simulink model "ForwardKinematic_YuMi"  (R2024a)
(part 17 of 23)

(2579692110316253*sin(q1R))/4503599627370496))/36893488147419103232 + sin(q2R)*((2579692110316253*cos(q1R))/4503599627370496 - (1917820484151683*sin(q1R))/18014398509481984)))/12259964326927110866866776217202473468949912977468817408 + (1764482024691522628700660907665*sin(q3R)*(cos(q2R)*((2579692110316253*cos(q1R))/4503599627370496 - (1917820484151683*sin(q1R))/18014398509481984) - (32968958366167862000829996477285*sin(q2R))/40564819207303340847894502572032 + (7514214926474921*sin(q2R)*((1917820484151683*cos(q1R))/18014398509481984 + (2579692110316253*sin(q1R))/4503599627370496))/36893488147419103232))/42535295865117307932921825928971026432 + (67682029681889335677290557259385*cos(q4R)*(cos(q3R)*(cos(q2R)*((2579692110316253*cos(q1R))/4503599627370496 - (1917820484151683*sin(q1R))/18014398509481984) - (32968958366167862000829996477285*sin(q2R))/40564819207303340847894502572032 + (7514214926474921*sin(q2R)*((1917820484151683*cos(q1R))/18014398509481984 + (2579692110316253*sin(q1R))/4503599627370496))/36893488147419103232) - (9007199067919185*sin(q3R)*((17274190877287359225804725738355*cos(q1R))/162259276829213363391578010288128 + (23235800371559029388956996013805*sin(q1R))/40564819207303340847894502572032 + 27504203825998033884751021716381/166153499473114484112975882535043072))/9007199254740992 + (7514214926474921*sin(q3R)*((32968958366167862000829996477285*cos(q2R))/40564819207303340847894502572032 - (7514214926474921*cos(q2R)*((1917820484151683*cos(q1R))/18014398509481984 + (2579692110316253*sin(q1R))/4503599627370496))/36893488147419103232 + sin(q2R)*((2579692110316253*cos(q1R))/4503599627370496 - (1917820484151683*sin(q1R))/18014398509481984)))/36893488147419103232))/332306998946228968225951765070086144))/16225927682921336339157801028812800 - (2436553109258773196144549622003023*cos(q6R)*(sin(q5R)*(((7514214926474921*cos(q4R))/36893488147419103232 + (4503599440548691*sin(q4R))/4503599627370496)*((9007199067919185*cos(q3R)*((17274190877287359225804725738355*cos(q1R))/162259276829213363391578010288128 + (23235800371559029388956996013805*sin(q1R))/40564819207303340847894502572032 + 27504203825998033884751021716381/166153499473114484112975882535043072))/9007199254740992 - (7514214926474921*cos(q3R)*((32968958366167862000829996477285*cos(q2R))/40564819207303340847894502572032 - (7514214926474921*cos(q2R)*((1917820484151683*cos(q1R))/18014398509481984 + (2579692110316253*sin(q1R))/4503599627370496))/36893488147419103232 + sin(q2R)*((2579692110316253*cos(q1R))/4503599627370496 - (1917820484151683*sin(q1R))/18014398509481984)))/36893488147419103232 + sin(q3R)*(cos(q2R)*((2579692110316253*cos(q1R))/4503599627370496 - (1917820484151683*sin(q1R))/18014398509481984) - (32968958366167862000829996477285*sin(q2R))/40564819207303340847894502572032 + (7514214926474921*sin(q2R)*((1917820484151683*cos(q1R))/18014398509481984 + (2579692110316253*sin(q1R))/4503599627370496))/36893488147419103232)) + (7514214926474921*sin(q4R)*(cos(q3R)*(cos(q2R)*((2579692110316253*cos(q1R))/4503599627370496 - (1917820484151683*sin(q1R))/18014398509481984) - (32968958366167862000829996477285*sin(q2R))/40564819207303340847894502572032 + (7514214926474921*sin(q2R)*((1917820484151683*cos(q1R))/18014398509481984 + (2579692110316253*sin(q1R))/4503599627370496))/36893488147419103232) - (9007199067919185*sin(q3R)*((17274190877287359225804725738355*cos(q1R))/162259276829213363391578010288128 + (23235800371559029388956996013805*sin(q1R))/40564819207303340847894502572032 + 27504203825998033884751021716381/166153499473114484112975882535043072))/9007199254740992 + (7514214926474921*sin(q3R)*((32968958366167862000829996477285*cos(q2R))/40564819207303340847894502572032 - (7514214926474921*cos(q2R)*((1917820484151683*cos(q1R))/18014398509481984 + (2579692110316253*sin(q1R))/4503599627370496))/36893488147419103232 + sin(q2R)*((2579692110316253*cos(q1R))/4503599627370496 - (1917820484151683*sin(q1R))/18014398509481984)))/36893488147419103232))/36893488147419103232) - (9007199067919185*cos(q5R)*((2115063383689692319117831580025*cos(q3R)*((17274190877287359225804725738355*cos(q1R))/162259276829213363391578010288128 + (23235800371559029388956996013805*sin(q1R))/40564819207303340847894502572032 + 27504203825998033884751021716381/166153499473114484112975882535043072))/10384593717069655257060992658440192 + (81129635049124235038645691064225*sin(q3R)*((17274190877287359225804725738355*cos(q1R))/162259276829213363391578010288128 + (23235800371559029388956996013805*sin(q1R))/40564819207303340847894502572032 + 27504203825998033884751021716381/166153499473114484112975882535043072))/81129638414606681695789005144064 - (1764482024691522628700660907665*cos(q3R)*((32968958366167862000829996477285*cos(q2R))/40564819207303340847894502572032 - (7514214926474921*cos(q2R)*((1917820484151683*cos(q1R))/18014398509481984 + (2579692110316253*sin(q1R))/4503599627370496))/36893488147419103232 + sin(q2R)*((2579692110316253*cos(q1R))/4503599627370496 - (1917820484151683*sin(q1R))/18014398509481984)))/42535295865117307932921825928971026432 - (9007199067919185*cos(q3R)*(cos(q2R)*((2579692110316253*cos(q1R))/4503599627370496 - (1917820484151683*sin(q1R))/18014398509481984) - (32968958366167862000829996477285*sin(q2R))/40564819207303340847894502572032 + (7514214926474921*sin(q2R)*((1917820484151683*cos(q1R))/18014398509481984 + (2579692110316253*sin(q1R))/4503599627370496))/36893488147419103232))/9007199254740992 - (67682029681889335677290557259385*sin(q3R)*((32968958366167862000829996477285*cos(q2R))/40564819207303340847894502572032 - (7514214926474921*cos(q2R)*((1917820484151683*cos(q1R))/18014398509481984 + (2579692110316253*sin(q1R))/4503599627370496))/36893488147419103232 + sin(q2R)*((2579692110316253*cos(q1R))/4503599627370496 - (1917820484151683*sin(q1R))/18014398509481984)))/332306998946228968225951765070086144 + (234819211581865*sin(q3R)*(cos(q2R)*((2579692110316253*cos(q1R))/4503599627370496 - (1917820484151683*sin(q1R))/18014398509481984) - (32968958366167862000829996477285*sin(q2R))/40564819207303340847894502572032 + (7514214926474921*sin(q2R)*((1917820484151683*cos(q1R))/18014398509481984 + (2579692110316253*sin(q1R))/4503599627370496))/36893488147419103232))/1152921504606846976))/9007199254740992 + (7514214926474921*cos(q5R)*(((4503599440548691*cos(q4R))/4503599627370496 - (7514214926474921*sin(q4R))/36893488147419103232)*((9007199067919185*cos(q3R)*((17274190877287359225804725738355*cos(q1R))/162259276829213363391578010288128 + (23235800371559029388956996013805*sin(q1R))/40564819207303340847894502572032 + 27504203825998033884751021716381/166153499473114484112975882535043072))/9007199254740992 - (7514214926474921*cos(q3R)*((32968958366167862000829996477285*cos(q2R))/40564819207303340847894502572032 - (7514214926474921*cos(q2R)*((1917820484151683*cos(q1R))/18014398509481984 + (2579692110316253*sin(q1R))/4503599627370496))/36893488147419103232 + sin(q2R)*((2579692110316253*cos(q1R))/4503599627370496 - (1917820484151683*sin(q1R))/18014398509481984)))/36893488147419103232 + sin(q3R)*(cos(q2R)*((2579692110316253*cos(q1R))/4503599627370496 - (1917820484151683*sin(q1R))/18014398509481984) - (32968958366167862000829996477285*sin(q2R))/40564819207303340847894502572032 + (7514214926474921*sin(q2R)*((1917820484151683*cos(q1R))/18014398509481984 + (2579692110316253*sin(q1R))/4503599627370496))/36893488147419103232)) + (7514214926474921*cos(q4R)*(cos(q3R)*(cos(q2R)*((2579692110316253*cos(q1R))/4503599627370496 - (1917820484151683*sin(q1R))/18014398509481984) - (32968958366167862000829996477285*sin(q2R))/40564819207303340847894502572032 + (7514214926474921*sin(q2R)*((1917820484151683*cos(q1R))/18014398509481984 + (2579692110316253*sin(q1R))/4503599627370496))/36893488147419103232) - (9007199067919185*sin(q3R)*((17274190877287359225804725738355*cos(q1R))/162259276829213363391578010288128 + (23235800371559029388956996013805*sin(q1R))/40564819207303340847894502572032 + 27504203825998033884751021716381/166153499473114484112975882535043072))/9007199254740992 + (7514214926474921*sin(q3R)*((32968958366167862000829996477285*cos(q2R))/40564819207303340847894502572032 - (7514214926474921*cos(q2R)*((1917820484151683*cos(q1R))/18014398509481984 + (2579692110316253*sin(q1R))/4503599627370496))/36893488147419103232 + sin(q2R)*((2579692110316253*cos(q1R))/4503599627370496 - (1917820484151683*sin(q1R))/18014398509481984)))/36893488147419103232))/36893488147419103232))/36893488147419103232))/332306998946228968225951765070086144000 - (48638874966763599*sin(q6R)*((15893040848161638993908057577265778144967053025*cos(q3R)*((17274190877287359225804725738355*cos(q1R))/162259276829213363391578010288128 + (23235800371559029388956996013805*sin(q1R))/40564819207303340847894502572032 + 27504203825998033884751021716381/166153499473114484112975882535043072))/383123885216472214589586756787577295904684780545900544 + (609625514665592237562888769449172969868262801225*sin(q3R)*((17274190877287359225804725738355*cos(q1R))/162259276829213363391578010288128 + (23235800371559029388956996013805*sin(q1R))/40564819207303340847894502572032 + 27504203825998033884751021716381/166153499473114484112975882535043072))/2993155353253689176481146537402947624255349848014848 + (9007199067919185*((4503599440548691*cos(q4R))/4503599627370496 - (7514214926474921*sin(q4R))/36893488147419103232)*((9007199067919185*cos(q3R)*((17274190877287359225804725738355*cos(q1R))/162259276829213363391578010288128 + (23235800371559029388956996013805*sin(q1R))/40564819207303340847894502572032 + 27504203825998033884751021716381/166153499473114484112975882535043072))/9007199254740992 - (7514214926474921*cos(q3R)*((32968958366167862000829996477285*cos(q2R))/40564819207303340847894502572032 - (7514214926474921*cos(q2R)*((1917820484151683*cos(q1R))/18014398509481984 + (2579692110316253*sin(q1R))/4503599627370496))/36893488147419103232 + sin(q2R)*((2579692110316253*cos(q1R))/4503599627370496 - (1917820484151683*sin(q1R))/18014398509481984)))/36893488147419103232 + sin(q3R)*(cos(q2R)*((2579692110316253*cos(q1R))/4503599627370496 - (1917820484151683*sin(q1R))/18014398509481984) - (32968958366167862000829996477285*sin(q2R))/40564819207303340847894502572032 + (7514214926474921*sin(q2R)*((1917820484151683*cos(q1R))/18014398509481984 + (2579692110316253*sin(q1R))/4503599627370496))/36893488147419103232)))/9007199254740992 - (13258697167433729449897784796786197386719169465*cos(q3R)*((32968958366167862000829996477285*cos(q2R))/40564819207303340847894502572032 - (7514214926474921*cos(q2R)*((1917820484151683*cos(q1R))/18014398509481984 + (2579692110316253*sin(q1R))/4503599627370496))/36893488147419103232 + sin(q2R)*((2579692110316253*cos(q1R))/4503599627370496 - (1917820484151683*sin(q1R))/18014398509481984)))/1569275433846670190958947355801916604025588861116008628224 - (67682029681889335677290557259385*cos(q3R)*(cos(q2R)*((2579692110316253*cos(q1R))/4503599627370496 - (1917820484151683*sin(q1R))/18014398509481984) - (32968958366167862000829996477285*sin(q2R))/40564819207303340847894502572032 + (7514214926474921*sin(q2R)*((1917820484151683*cos(q1R))/18014398509481984 + (2579692110316253*sin(q1R))/4503599627370496))/36893488147419103232))/332306998946228968225951765070086144 - (508577317689771495245073589786522929324694383585*sin(q3R)*((32968958366167862000829996477285*cos(q2R))/40564819207303340847894502572032 - (7514214926474921*cos(q2R)*((1917820484151683*cos(q1R))/18014398509481984 + (2579692110316253*sin(q1R))/4503599627370496))/36893488147419103232 + sin(q2R)*((2579692110316253*cos(q1R))/4503599627370496 - (1917820484151683*sin(q1R))/18014398509481984)))/12259964326927110866866776217202473468949912977468817408 + (1764482024691522628700660907665*sin(q3R)*(cos(q2R)*((2579692110316253*cos(q1R))/4503599627370496 - (1917820484151683*sin(q1R))/18014398509481984) - (32968958366167862000829996477285*sin(q2R))/40564819207303340847894502572032 + (7514214926474921*sin(q2R)*((1917820484151683*cos(q1R))/18014398509481984 + (2579692110316253*sin(q1R))/4503599627370496))/36893488147419103232))/42535295865117307932921825928971026432 + (67682029681889335677290557259385*cos(q4R)*(cos(q3R)*(cos(q2R)*((2579692110316253*cos(q1R))/4503599627370496 - (1917820484151683*sin(q1R))/18014398509481984) - (32968958366167862000829996477285*sin(q2R))/40564819207303340847894502572032 + (7514214926474921*sin(q2R)*((1917820484151683*cos(q1R))/18014398509481984 + (2579692110316253*sin(q1R))/4503599627370496))/36893488147419103232) - (9007199067919185*sin(q3R)*((17274190877287359225804725738355*cos(q1R))/162259276829213363391578010288128 + (23235800371559029388956996013805*sin(q1R))/40564819207303340847894502572032 + 27504203825998033884751021716381/166153499473114484112975882535043072))/9007199254740992 + (7514214926474921*sin(q3R)*((32968958366167862000829996477285*cos(q2R))/40564819207303340847894502572032 - (7514214926474921*cos(q2R)*((1917820484151683*cos(q1R))/18014398509481984 + (2579692110316253*sin(q1R))/4503599627370496))/36893488147419103232 + sin(q2R)*((2579692110316253*cos(q1R))/4503599627370496 - (1917820484151683*sin(q1R))/18014398509481984)))/36893488147419103232))/332306998946228968225951765070086144))/1801439850948198400 - (27*cos(q6R)*(cos(q5R)*(((7514214926474921*cos(q4R))/36893488147419103232 + (4503599440548691*sin(q4R))/4503599627370496)*((9007199067919185*cos(q3R)*((17274190877287359225804725738355*cos(q1R))/162259276829213363391578010288128 + (23235800371559029388956996013805*sin(q1R))/40564819207303340847894502572032 + 27504203825998033884751021716381/166153499473114484112975882535043072))/9007199254740992 - (7514214926474921*cos(q3R)*((32968958366167862000829996477285*cos(q2R))/40564819207303340847894502572032 - (7514214926474921*cos(q2R)*((1917820484151683*cos(q1R))/18014398509481984 + (2579692110316253*sin(q1R))/4503599627370496))/36893488147419103232 + sin(q2R)*((2579692110316253*cos(q1R))/4503599627370496 - (1917820484151683*sin(q1R))/18014398509481984)))/36893488147419103232 + sin(q3R)*(cos(q2R)*((2579692110316253*cos(q1R))/4503599627370496 - (1917820484151683*sin(q1R))/18014398509481984) - (32968958366167862000829996477285*sin(q2R))/40564819207303340847894502572032 + (7514214926474921*sin(q2R)*((1917820484151683*cos(q1R))/18014398509481984 + (2579692110316253*sin(q1R))/4503599627370496))/36893488147419103232)) + (7514214926474921*sin(q4R)*(cos(q3R)*(cos(q2R)*((2579692110316253*cos(q1R))/4503599627370496 - (1917820484151683*sin(q1R))/18014398509481984) - (32968958366167862000829996477285*sin(q2R))/40564819207303340847894502572032 + (7514214926474921*sin(q2R)*((1917820484151683*cos(q1R))/18014398509481984 + (2579692110316253*sin(q1R))/4503599627370496))/36893488147419103232) - (9007199067919185*sin(q3R)*((17274190877287359225804725738355*cos(q1R))/162259276829213363391578010288128 + (23235800371559029388956996013805*sin(q1R))/40564819207303340847894502572032 + 27504203825998033884751021716381/166153499473114484112975882535043072))/9007199254740992 + (7514214926474921*sin(q3R)*((32968958366167862000829996477285*cos(q2R))/40564819207303340847894502572032 - (7514214926474921*cos(q2R)*((1917820484151683*cos(q1R))/18014398509481984 + (2579692110316253*sin(q1R))/4503599627370496))/36893488147419103232 + sin(q2R)*((2579692110316253*cos(q1R))/4503599627370496 - (1917820484151683*sin(q1R))/18014398509481984)))/36893488147419103232))/36893488147419103232) - (7514214926474921*sin(q5R)*(((4503599440548691*cos(q4R))/4503599627370496 - (7514214926474921*sin(q4R))/36893488147419103232)*((9007199067919185*cos(q3R)*((17274190877287359225804725738355*cos(q1R))/162259276829213363391578010288128 + (23235800371559029388956996013805*sin(q1R))/40564819207303340847894502572032 + 27504203825998033884751021716381/166153499473114484112975882535043072))/9007199254740992 - (7514214926474921*cos(q3R)*((32968958366167862000829996477285*cos(q2R))/40564819207303340847894502572032 - (7514214926474921*cos(q2R)*((1917820484151683*cos(q1R))/18014398509481984 + (2579692110316253*sin(q1R))/4503599627370496))/36893488147419103232 + sin(q2R)*((2579692110316253*cos(q1R))/4503599627370496 - (1917820484151683*sin(q1R))/18014398509481984)))/36893488147419103232 + sin(q3R)*(cos(q2R)*((2579692110316253*cos(q1R))/4503599627370496 - (1917820484151683*sin(q1R))/18014398509481984) - (32968958366167862000829996477285*sin(q2R))/40564819207303340847894502572032 + (7514214926474921*sin(q2R)*((1917820484151683*cos(q1R))/18014398509481984 + (2579692110316253*sin(q1R))/4503599627370496))/36893488147419103232)) + (7514214926474921*cos(q4R)*(cos(q3R)*(cos(q2R)*((2579692110316253*cos(q1R))/4503599627370496 - (1917820484151683*sin(q1R))/18014398509481984) - (32968958366167862000829996477285*sin(q2R))/40564819207303340847894502572032 + (7514214926474921*sin(q2R)*((1917820484151683*cos(q1R))/18014398509481984 + (2579692110316253*sin(q1R))/4503599627370496))/36893488147419103232) - (9007199067919185*sin(q3R)*((17274190877287359225804725738355*cos(q1R))/162259276829213363391578010288128 + (23235800371559029388956996013805*sin(q1R))/40564819207303340847894502572032 + 27504203825998033884751021716381/166153499473114484112975882535043072))/9007199254740992 + (7514214926474921*sin(q3R)*((32968958366167862000829996477285*cos(q2R))/40564819207303340847894502572032 - (7514214926474921*cos(q2R)*((1917820484151683*cos(q1R))/18014398509481984 + (2579692110316253*sin(q1R))/4503599627370496))/36893488147419103232 + sin(q2R)*((2579692110316253*cos(q1R))/4503599627370496 - (1917820484151683*sin(q1R))/18014398509481984)))/36893488147419103232))/36893488147419103232))/36893488147419103232 + (9007199067919185*sin(q5R)*((2115063383689692319117831580025*cos(q3R)*((17274190877287359225804725738355*cos(q1R))/162259276829213363391578010288128 + (23235800371559029388956996013805*sin(q1R))/40564819207303340847894502572032 + 27504203825998033884751021716381/166153499473114484112975882535043072))/10384593717069655257060992658440192 + (81129635049124235038645691064225*sin(q3R)*((17274190877287359225804725738355*cos(q1R))/162259276829213363391578010288128 + (23235800371559029388956996013805*sin(q1R))/40564819207303340847894502572032 + 27504203825998033884751021716381/166153499473114484112975882535043072))/81129638414606681695789005144064 - (1764482024691522628700660907665*cos(q3R)*((32968958366167862000829996477285*cos(q2R))/40564819207303340847894502572032 - (7514214926474921*cos(q2R)*((1917820484151683*cos(q1R))/18014398509481984 + (2579692110316253*sin(q1R))/4503599627370496))/36893488147419103232 + sin(q2R)*((2579692110316253*cos(q1R))/4503599627370496 - (1917820484151683*sin(q1R))/18014398509481984)))/42535295865117307932921825928971026432 - (9007199067919185*cos(q3R)*(cos(q2R)*((2579692110316253*cos(q1R))/4503599627370496 - (1917820484151683*sin(q1R))/18014398509481984) - (32968958366167862000829996477285*sin(q2R))/40564819207303340847894502572032 + (7514214926474921*sin(q2R)*((1917820484151683*cos(q1R))/18014398509481984 + (2579692110316253*sin(q1R))/4503599627370496))/36893488147419103232))/9007199254740992 - (67682029681889335677290557259385*sin(q3R)*((32968958366167862000829996477285*cos(q2R))/40564819207303340847894502572032 - (7514214926474921*cos(q2R)*((1917820484151683*cos(q1R))/18014398509481984 + (2579692110316253*sin(q1R))/4503599627370496))/36893488147419103232 + sin(q2R)*((2579692110316253*cos(q1R))/4503599627370496 - (1917820484151683*sin(q1R))/18014398509481984)))/332306998946228968225951765070086144 + (234819211581865*sin(q3R)*(cos(q2R)*((2579692110316253*cos(q1R))/4503599627370496 - (1917820484151683*sin(q1R))/18014398509481984) - (32968958366167862000829996477285*sin(q2R))/40564819207303340847894502572032 + (7514214926474921*sin(q2R)*((1917820484151683*cos(q1R))/18014398509481984 + (2579692110316253*sin(q1R))/4503599627370496))/36893488147419103232))/1152921504606846976))/9007199254740992))/1000 - (202883803014822867*sin(q6R)*(sin(q5R)*(((7514214926474921*cos(q4R))/36893488147419103232 + (4503599440548691*sin(q4R))/4503599627370496)*((9007199067919185*cos(q3R)*((17274190877287359225804725738355*cos(q1R))/162259276829213363391578010288128 + (23235800371559029388956996013805*sin(q1R))/40564819207303340847894502572032 + 27504203825998033884751021716381/166153499473114484112975882535043072))/9007199254740992 - (7514214926474921*cos(q3R)*((32968958366167862000829996477285*cos(q2R))/40564819207303340847894502572032 - (7514214926474921*cos(q2R)*((1917820484151683*cos(q1R))/18014398509481984 + (2579692110316253*sin(q1R))/4503599627370496))/36893488147419103232 + sin(q2R)*((2579692110316253*cos(q1R))/4503599627370496 - (1917820484151683*sin(q1R))/18014398509481984)))/36893488147419103232 + sin(q3R)*(cos(q2R)*((2579692110316253*cos(q1R))/4503599627370496 - (1917820484151683*sin(q1R))/18014398509481984) - (32968958366167862000829996477285*sin(q2R))/40564819207303340847894502572032 + (7514214926474921*sin(q2R)*((1917820484151683*cos(q1R))/18014398509481984 + (2579692110316253*sin(q1R))/4503599627370496))/36893488147419103232)) + (7514214926474921*sin(q4R)*(cos(q3R)*(cos(q2R)*((2579692110316253*cos(q1R))/4503599627370496 - (1917820484151683*sin(q1R))/18014398509481984) - (32968958366167862000829996477285*sin(q2R))/40564819207303340847894502572032 + (7514214926474921*sin(q2R)*((1917820484151683*cos(q1R))/18014398509481984 + (2579692110316253*sin(q1R))/4503599627370496))/36893488147419103232) - (9007199067919185*sin(q3R)*((17274190877287359225804725738355*cos(q1R))/162259276829213363391578010288128 + (23235800371559029388956996013805*sin(q1R))/40564819207303340847894502572032 + 27504203825998033884751021716381/166153499473114484112975882535043072))/9007199254740992 + (7514214926474921*sin(q3R)*((32968958366167862000829996477285*cos(q2R))/40564819207303340847894502572032 - (7514214926474921*cos(q2R)*((1917820484151683*cos(q1R))/18014398509481984 + (2579692110316253*sin(q1R))/4503599627370496))/36893488147419103232 + sin(q2R)*((2579692110316253*cos(q1R))/4503599627370496 - (1917820484151683*sin(q1R))/18014398509481984)))/36893488147419103232))/36893488147419103232) - (9007199067919185*cos(q5R)*((2115063383689692319117831580025*cos(q3R)*((17274190877287359225804725738355*cos(q1R))/162259276829213363391578010288128 + (23235800371559029388956996013805*sin(q1R))/40564819207303340847894502572032 + 27504203825998033884751021716381/166153499473114484112975882535043072))/10384593717069655257060992658440192 + (81129635049124235038645691064225*sin(q3R)*((17274190877287359225804725738355*cos(q1R))/162259276829213363391578010288128 + (23235800371559029388956996013805*sin(q1R))/40564819207303340847894502572032 + 27504203825998033884751021716381/166153499473114484112975882535043072))/81129638414606681695789005144064 - (1764482024691522628700660907665*cos(q3R)*((32968958366167862000829996477285*cos(q2R))/40564819207303340847894502572032 - (7514214926474921*cos(q2R)*((1917820484151683*cos(q1R))/18014398509481984 + (2579692110316253*sin(q1R))/4503599627370496))/36893488147419103232 + sin(q2R)*((2579692110316253*cos(q1R))/4503599627370496 - (1917820484151683*sin(q1R))/18014398509481984)))/42535295865117307932921825928971026432 - (9007199067919185*cos(q3R)*(cos(q2R)*((2579692110316253*cos(q1R))/4503599627370496 - (1917820484151683*sin(q1R))/18014398509481984) - (32968958366167862000829996477285*sin(q2R))/40564819207303340847894502572032 + (7514214926474921*sin(q2R)*((1917820484151683*cos(q1R))/18014398509481984 + (2579692110316253*sin(q1R))/4503599627370496))/36893488147419103232))/9007199254740992 - (67682029681889335677290557259385*sin(q3R)*((32968958366167862000829996477285*cos(q2R))/40564819207303340847894502572032 - (7514214926474921*cos(q2R)*((1917820484151683*cos(q1R))/18014398509481984 + (2579692110316253*sin(q1R))/4503599627370496))/36893488147419103232 + sin(q2R)*((2579692110316253*cos(q1R))/4503599627370496 - (1917820484151683*sin(q1R))/18014398509481984)))/332306998946228968225951765070086144 + (234819211581865*sin(q3R)*(cos(q2R)*((2579692110316253*cos(q1R))/4503599627370496 - (1917820484151683*sin(q1R))/18014398509481984) - (32968958366167862000829996477285*sin(q2R))/40564819207303340847894502572032 + (7514214926474921*sin(q2R)*((1917820484151683*cos(q1R))/18014398509481984 + (2579692110316253*sin(q1R))/4503599627370496))/36893488147419103232))/1152921504606846976))/9007199254740992 + (7514214926474921*cos(q5R)*(((4503599440548691*cos(q4R))/4503599627370496 - (7514214926474921*sin(q4R))/36893488147419103232)*((9007199067919185*cos(q3R)*((17274190877287359225804725738355*cos(q1R))/162259276829213363391578010288128 + (23235800371559029388956996013805*sin(q1R))/40564819207303340847894502572032 + 27504203825998033884751021716381/166153499473114484112975882535043072))/9007199254740992 - (7514214926474921*cos(q3R)*((32968958366167862000829996477285*cos(q2R))/40564819207303340847894502572032 - (7514214926474921*cos(q2R)*((1917820484151683*cos(q1R))/18014398509481984 + (2579692110316253*sin(q1R))/4503599627370496))/36893488147419103232 + sin(q2R)*((2579692110316253*cos(q1R))/4503599627370496 - (1917820484151683*sin(q1R))/18014398509481984)))/36893488147419103232 + sin(q3R)*(cos(q2R)*((2579692110316253*cos(q1R))/4503599627370496 - (1917820484151683*sin(q1R))/18014398509481984) - (32968958366167862000829996477285*sin(q2R))/40564819207303340847894502572032 + (7514214926474921*sin(q2R)*((1917820484151683*cos(q1R))/18014398509481984 + (2579692110316253*sin(q1R))/4503599627370496))/36893488147419103232)) + (7514214926474921*cos(q4R)*(cos(q3R)*(cos(q2R)*((2579692110316253*cos(q1R))/4503599627370496 - (1917820484151683*sin(q1R))/18014398509481984) - (32968958366167862000829996477285*sin(q2R))/40564819207303340847894502572032 + (7514214926474921*sin(q2R)*((1917820484151683*cos(q1R))/18014398509481984 + (2579692110316253*sin(q1R))/4503599627370496))/36893488147419103232) - (9007199067919185*sin(q3R)*((17274190877287359225804725738355*cos(q1R))/162259276829213363391578010288128 + (23235800371559029388956996013805*sin(q1R))/40564819207303340847894502572032 + 27504203825998033884751021716381/166153499473114484112975882535043072))/9007199254740992 + (7514214926474921*sin(q3R)*((32968958366167862000829996477285*cos(q2R))/40564819207303340847894502572032 - (7514214926474921*cos(q2R)*((1917820484151683*cos(q1R))/18014398509481984 + (2579692110316253*sin(q1R))/4503599627370496))/36893488147419103232 + sin(q2R)*((2579692110316253*cos(q1R))/4503599627370496 - (1917820484151683*sin(q1R))/18014398509481984)))/36893488147419103232))/36893488147419103232))/36893488147419103232))/36893488147419103232000 - (610321541873521657855151997354401418608858870661075444886782706002880706727*cos(q4R)*(cos(q3R)*(cos(q2R)*((2579692110316253*cos(q1R))/4503599627370496 - (1917820484151683*sin(q1R))/18014398509481984) - (32968958366167862000829996477285*sin(q2R))/40564819207303340847894502572032 + (7514214926474921*sin(q2R)*((1917820484151683*cos(q1R))/18014398509481984 + (2579692110316253*sin(q1R))/4503599627370496))/36893488147419103232) - (9007199067919185*sin(q3R)*((17274190877287359225804725738355*cos(q1R))/162259276829213363391578010288128 + (23235800371559029388956996013805*sin(q1R))/40564819207303340847894502572032 + 27504203825998033884751021716381/166153499473114484112975882535043072))/9007199254740992 + (7514214926474921*sin(q3R)*((32968958366167862000829996477285*cos(q2R))/40564819207303340847894502572032 - (7514214926474921*cos(q2R)*((1917820484151683*cos(q1R))/18014398509481984 + (2579692110316253*sin(q1R))/4503599627370496))/36893488147419103232 + sin(q2R)*((2579692110316253*cos(q1R))/4503599627370496 - (1917820484151683*sin(q1R))/18014398509481984)))/36893488147419103232))/11307821214581659709333104004754678501295896940003961331978279688272766566400000 + (324259171862923063*sin(q6R)*(cos(q5R)*(((7514214926474921*cos(q4R))/36893488147419103232 + (4503599440548691*sin(q4R))/4503599627370496)*((9007199067919185*cos(q3R)*((17274190877287359225804725738355*cos(q1R))/162259276829213363391578010288128 + (23235800371559029388956996013805*sin(q1R))/40564819207303340847894502572032 + 27504203825998033884751021716381/166153499473114484112975882535043072))/9007199254740992 - (7514214926474921*cos(q3R)*((32968958366167862000829996477285*cos(q2R))/40564819207303340847894502572032 - (7514214926474921*cos(q2R)*((1917820484151683*cos(q1R))/18014398509481984 + (2579692110316253*sin(q1R))/4503599627370496))/36893488147419103232 + sin(q2R)*((2579692110316253*cos(q1R))/4503599627370496 - (1917820484151683*sin(q1R))/18014398509481984)))/36893488147419103232 + sin(q3R)*(cos(q2R)*((2579692110316253*cos(q1R))/4503599627370496 - (1917820484151683*sin(q1R))/18014398509481984) - (32968958366167862000829996477285*sin(q2R))/40564819207303340847894502572032 + (7514214926474921*sin(q2R)*((1917820484151683*cos(q1R))/18014398509481984 + (2579692110316253*sin(q1R))/4503599627370496))/36893488147419103232)) + (7514214926474921*sin(q4R)*(cos(q3R)*(cos(q2R)*((2579692110316253*cos(q1R))/4503599627370496 - (1917820484151683*sin(q1R))/18014398509481984) - (32968958366167862000829996477285*sin(q2R))/40564819207303340847894502572032 + (7514214926474921*sin(q2R)*((1917820484151683*cos(q1R))/18014398509481984 + (2579692110316253*sin(q1R))/4503599627370496))/36893488147419103232) - (9007199067919185*sin(q3R)*((17274190877287359225804725738355*cos(q1R))/162259276829213363391578010288128 + (23235800371559029388956996013805*sin(q1R))/40564819207303340847894502572032 + 27504203825998033884751021716381/166153499473114484112975882535043072))/9007199254740992 + (7514214926474921*sin(q3R)*((32968958366167862000829996477285*cos(q2R))/40564819207303340847894502572032 - (7514214926474921*cos(q2R)*((1917820484151683*cos(q1R))/18014398509481984 + (2579692110316253*sin(q1R))/4503599627370496))/36893488147419103232 + sin(q2R)*((2579692110316253*cos(q1R))/4503599627370496 - (1917820484151683*sin(q1R))/18014398509481984)))/36893488147419103232))/36893488147419103232) - (7514214926474921*sin(q5R)*(((4503599440548691*cos(q4R))/4503599627370496 - (7514214926474921*sin(q4R))/36893488147419103232)*((9007199067919185*cos(q3R)*((17274190877287359225804725738355*cos(q1R))/162259276829213363391578010288128 + (23235800371559029388956996013805*sin(q1R))/40564819207303340847894502572032 + 27504203825998033884751021716381/166153499473114484112975882535043072))/9007199254740992 - (7514214926474921*cos(q3R)*((32968958366167862000829996477285*cos(q2R))/40564819207303340847894502572032 - (7514214926474921*cos(q2R)*((1917820484151683*cos(q1R))/18014398509481984 + (2579692110316253*sin(q1R))/4503599627370496))/36893488147419103232 + sin(q2R)*((2579692110316253*cos(q1R))/4503599627370496 - (1917820484151683*sin(q1R))/18014398509481984)))/36893488147419103232 + sin(q3R)*(cos(q2R)*((2579692110316253*cos(q1R))/4503599627370496 - (1917820484151683*sin(q1R))/18014398509481984) - (32968958366167862000829996477285*sin(q2R))/40564819207303340847894502572032 + (7514214926474921*sin(q2R)*((1917820484151683*cos(q1R))/18014398509481984 + (2579692110316253*sin(q1R))/4503599627370496))/36893488147419103232)) + (7514214926474921*cos(q4R)*(cos(q3R)*(cos(q2R)*((2579692110316253*cos(q1R))/4503599627370496 - (1917820484151683*sin(q1R))/18014398509481984) - (32968958366167862000829996477285*sin(q2R))/40564819207303340847894502572032 + (7514214926474921*sin(q2R)*((1917820484151683*cos(q1R))/18014398509481984 + (2579692110316253*sin(q1R))/4503599627370496))/36893488147419103232) - (9007199067919185*sin(q3R)*((17274190877287359225804725738355*cos(q1R))/162259276829213363391578010288128 + (23235800371559029388956996013805*sin(q1R))/40564819207303340847894502572032 + 27504203825998033884751021716381/166153499473114484112975882535043072))/9007199254740992 + (7514214926474921*sin(q3R)*((32968958366167862000829996477285*cos(q2R))/40564819207303340847894502572032 - (7514214926474921*cos(q2R)*((1917820484151683*cos(q1R))/18014398509481984 + (2579692110316253*sin(q1R))/4503599627370496))/36893488147419103232 + sin(q2R)*((2579692110316253*cos(q1R))/4503599627370496 - (1917820484151683*sin(q1R))/18014398509481984)))/36893488147419103232))/36893488147419103232))/36893488147419103232 + (9007199067919185*sin(q5R)*((2115063383689692319117831580025*cos(q3R)*((17274190877287359225804725738355*cos(q1R))/162259276829213363391578010288128 + (23235800371559029388956996013805*sin(q1R))/40564819207303340847894502572032 + 27504203825998033884751021716381/166153499473114484112975882535043072))/10384593717069655257060992658440192 + (81129635049124235038645691064225*sin(q3R)*((17274190877287359225804725738355*cos(q1R))/162259276829213363391578010288128 + (23235800371559029388956996013805*sin(q1R))/40564819207303340847894502572032 + 27504203825998033884751021716381/166153499473114484112975882535043072))/81129638414606681695789005144064 - (1764482024691522628700660907665*cos(q3R)*((32968958366167862000829996477285*cos(q2R))/40564819207303340847894502572032 - (7514214926474921*cos(q2R)*((1917820484151683*cos(q1R))/18014398509481984 + (2579692110316253*sin(q1R))/4503599627370496))/36893488147419103232 + sin(q2R)*((2579692110316253*cos(q1R))/4503599627370496 - (1917820484151683*sin(q1R))/18014398509481984)))/42535295865117307932921825928971026432 - (9007199067919185*cos(q3R)*(cos(q2R)*((2579692110316253*cos(q1R))/4503599627370496 - (1917820484151683*sin(q1R))/18014398509481984) - (32968958366167862000829996477285*sin(q2R))/40564819207303340847894502572032 + (7514214926474921*sin(q2R)*((1917820484151683*cos(q1R))/18014398509481984 + (2579692110316253*sin(q1R))/4503599627370496))/36893488147419103232))/9007199254740992 - (67682029681889335677290557259385*sin(q3R)*((32968958366167862000829996477285*cos(q2R))/40564819207303340847894502572032 - (7514214926474921*cos(q2R)*((1917820484151683*cos(q1R))/18014398509481984 + (2579692110316253*sin(q1R))/4503599627370496))/36893488147419103232 + sin(q2R)*((2579692110316253*cos(q1R))/4503599627370496 - (1917820484151683*sin(q1R))/18014398509481984)))/332306998946228968225951765070086144 + (234819211581865*sin(q3R)*(cos(q2R)*((2579692110316253*cos(q1R))/4503599627370496 - (1917820484151683*sin(q1R))/18014398509481984) - (32968958366167862000829996477285*sin(q2R))/40564819207303340847894502572032 + (7514214926474921*sin(q2R)*((1917820484151683*cos(q1R))/18014398509481984 + (2579692110316253*sin(q1R))/4503599627370496))/36893488147419103232))/1152921504606846976))/9007199254740992))/9007199254740992000 - (608651409044468601*sin(q4R)*(cos(q3R)*(cos(q2R)*((2579692110316253*cos(q1R))/4503599627370496 - (1917820484151683*sin(q1R))/18014398509481984) - (32968958366167862000829996477285*sin(q2R))/40564819207303340847894502572032 + (7514214926474921*sin(q2R)*((1917820484151683*cos(q1R))/18014398509481984 + (2579692110316253*sin(q1R))/4503599627370496))/36893488147419103232) - (9007199067919185*sin(q3R)*((17274190877287359225804725738355*cos(q1R))/162259276829213363391578010288128 + (23235800371559029388956996013805*sin(q1R))/40564819207303340847894502572032 + 27504203825998033884751021716381/166153499473114484112975882535043072))/9007199254740992 + (7514214926474921*sin(q3R)*((32968958366167862000829996477285*cos(q2R))/40564819207303340847894502572032 - (7514214926474921*cos(q2R)*((1917820484151683*cos(q1R))/18014398509481984 + (2579692110316253*sin(q1R))/4503599627370496))/36893488147419103232 + sin(q2R)*((2579692110316253*cos(q1R))/4503599627370496 - (1917820484151683*sin(q1R))/18014398509481984)))/36893488147419103232))/73786976294838206464000 + (712008244765680093343103025701132101054572137019*cos(q5R)*(((4503599440548691*cos(q4R))/4503599627370496 - (7514214926474921*sin(q4R))/36893488147419103232)*((9007199067919185*cos(q3R)*((17274190877287359225804725738355*cos(q1R))/162259276829213363391578010288128 + (23235800371559029388956996013805*sin(q1R))/40564819207303340847894502572032 + 27504203825998033884751021716381/166153499473114484112975882535043072))/9007199254740992 - (7514214926474921*cos(q3R)*((32968958366167862000829996477285*cos(q2R))/40564819207303340847894502572032 - (7514214926474921*cos(q2R)*((1917820484151683*cos(q1R))/18014398509481984 + (2579692110316253*sin(q1R))/4503599627370496))/36893488147419103232 + sin(q2R)*((2579692110316253*cos(q1R))/4503599627370496 - (1917820484151683*sin(q1R))/18014398509481984)))/36893488147419103232 + sin(q3R)*(cos(q2R)*((2579692110316253*cos(q1R))/4503599627370496 - (1917820484151683*sin(q1R))/18014398509481984) - (32968958366167862000829996477285*sin(q2R))/40564819207303340847894502572032 + (7514214926474921*sin(q2R)*((1917820484151683*cos(q1R))/18014398509481984 + (2579692110316253*sin(q1R))/4503599627370496))/36893488147419103232)) + (7514214926474921*cos(q4R)*(cos(q3R)*(cos(q2R)*((2579692110316253*cos(q1R))/4503599627370496 - (1917820484151683*sin(q1R))/18014398509481984) - (32968958366167862000829996477285*sin(q2R))/40564819207303340847894502572032 + (7514214926474921*sin(q2R)*((1917820484151683*cos(q1R))/18014398509481984 + (2579692110316253*sin(q1R))/4503599627370496))/36893488147419103232) - (9007199067919185*sin(q3R)*((17274190877287359225804725738355*cos(q1R))/162259276829213363391578010288128 + (23235800371559029388956996013805*sin(q1R))/40564819207303340847894502572032 + 27504203825998033884751021716381/166153499473114484112975882535043072))/9007199254740992 + (7514214926474921*sin(q3R)*((32968958366167862000829996477285*cos(q2R))/40564819207303340847894502572032 - (7514214926474921*cos(q2R)*((1917820484151683*cos(q1R))/18014398509481984 + (2579692110316253*sin(q1R))/4503599627370496))/36893488147419103232 + sin(q2R)*((2579692110316253*cos(q1R))/4503599627370496 - (1917820484151683*sin(q1R))/18014398509481984)))/36893488147419103232))/36893488147419103232))/2451992865385422173373355243440494693789982595493763481600, (81*((4503599440548691*cos(q4R))/4503599627370496 - (7514214926474921*sin(q4R))/36893488147419103232)*(cos(q3R)*(cos(q2R)*((2579692110316253*cos(q1R))/4503599627370496 - (1917820484151683*sin(q1R))/18014398509481984) - (32968958366167862000829996477285*sin(q2R))/40564819207303340847894502572032 + (7514214926474921*sin(q2R)*((1917820484151683*cos(q1R))/18014398509481984 + (2579692110316253*sin(q1R))/4503599627370496))/36893488147419103232) - (9007199067919185*sin(q3R)*((17274190877287359225804725738355*cos(q1R))/162259276829213363391578010288128 + (23235800371559029388956996013805*sin(q1R))/40564819207303340847894502572032 + 27504203825998033884751021716381/166153499473114484112975882535043072))/9007199254740992 + (7514214926474921*sin(q3R)*((32968958366167862000829996477285*cos(q2R))/40564819207303340847894502572032 - (7514214926474921*cos(q2R)*((1917820484151683*cos(q1R))/18014398509481984 + (2579692110316253*sin(q1R))/4503599627370496))/36893488147419103232 + sin(q2R)*((2579692110316253*cos(q1R))/4503599627370496 - (1917820484151683*sin(q1R))/18014398509481984)))/36893488147419103232))/2000 - (81222263116692158804177042061221826384594597321566869716687*((7514214926474921*cos(q4R))/36893488147419103232 + (4503599440548691*sin(q4R))/4503599627370496)*(cos(q3R)*(cos(q2R)*((2579692110316253*cos(q1R))/4503599627370496 - (1917820484151683*sin(q1R))/18014398509481984) - (32968958366167862000829996477285*sin(q2R))/40564819207303340847894502572032 + (7514214926474921*sin(q2R)*((1917820484151683*cos(q1R))/18014398509481984 + (2579692110316253*sin(q1R))/4503599627370496))/36893488147419103232) - (9007199067919185*sin(q3R)*((17274190877287359225804725738355*cos(q1R))/162259276829213363391578010288128 + (23235800371559029388956996013805*sin(q1R))/40564819207303340847894502572032 + 27504203825998033884751021716381/166153499473114484112975882535043072))/9007199254740992 + (7514214926474921*sin(q3R)*((32968958366167862000829996477285*cos(q2R))/40564819207303340847894502572032 - (7514214926474921*cos(q2R)*((1917820484151683*cos(q1R))/18014398509481984 + (2579692110316253*sin(q1R))/4503599627370496))/36893488147419103232 + sin(q2R)*((2579692110316253*cos(q1R))/4503599627370496 - (1917820484151683*sin(q1R))/18014398509481984)))/36893488147419103232))/306499108173177771671669405430061836723747824436720435200000 - (584133382113593486367040631332731*cos(q6R)*((9007199067919185*((7514214926474921*cos(q4R))/36893488147419103232 + (4503599440548691*sin(q4R))/4503599627370496)*(cos(q3R)*(cos(q2R)*((2579692110316253*cos(q1R))/4503599627370496 - (1917820484151683*sin(q1R))/18014398509481984) - (32968958366167862000829996477285*sin(q2R))/40564819207303340847894502572032 + (7514214926474921*sin(q2R)*((1917820484151683*cos(q1R))/18014398509481984 + (2579692110316253*sin(q1R))/4503599627370496))/36893488147419103232) - (9007199067919185*sin(q3R)*((17274190877287359225804725738355*cos(q1R))/162259276829213363391578010288128 + (23235800371559029388956996013805*sin(q1R))/40564819207303340847894502572032 + 27504203825998033884751021716381/166153499473114484112975882535043072))/9007199254740992 + (7514214926474921*sin(q3R)*((32968958366167862000829996477285*cos(q2R))/40564819207303340847894502572032 - (7514214926474921*cos(q2R)*((1917820484151683*cos(q1R))/18014398509481984 + (2579692110316253*sin(q1R))/4503599627370496))/36893488147419103232 + sin(q2R)*((2579692110316253*cos(q1R))/4503599627370496 - (1917820484151683*sin(q1R))/18014398509481984)))/36893488147419103232))/9007199254740992 - (67682029681889335677290557259385*sin(q4R)*((9007199067919185*cos(q3R)*((17274190877287359225804725738355*cos(q1R))/162259276829213363391578010288128 + (23235800371559029388956996013805*sin(q1R))/40564819207303340847894502572032 + 27504203825998033884751021716381/166153499473114484112975882535043072))/9007199254740992 - (7514214926474921*cos(q3R)*((32968958366167862000829996477285*cos(q2R))/40564819207303340847894502572032 - (7514214926474921*cos(q2R)*((1917820484151683*cos(q1R))/18014398509481984 + (2579692110316253*sin(q1R))/4503599627370496))/36893488147419103232 + sin(q2R)*((2579692110316253*cos(q1R))/4503599627370496 - (1917820484151683*sin(q1R))/18014398509481984)))/36893488147419103232 + sin(q3R)*(cos(q2R)*((2579692110316253*cos(q1R))/4503599627370496 - (1917820484151683*sin(q1R))/18014398509481984) - (32968958366167862000829996477285*sin(q2R))/40564819207303340847894502572032 + (7514214926474921*sin(q2R)*((1917820484151683*cos(q1R))/18014398509481984 + (2579692110316253*sin(q1R))/4503599627370496))/36893488147419103232)))/332306998946228968225951765070086144 + (9007199067919185*((9007199067919185*cos(q4R))/9007199254740992 - (234819211581865*sin(q4R))/1152921504606846976)*((129801982932889585091297864435361917839115294955*cos(q1R))/5986310706507378352962293074805895248510699696029696 + (296957971066013582975066703729047659005068212725*cos(q2R))/365375409332725729550921208179070754913983135744 + (174598797980560374072834504815488878557302284405*sin(q1R))/1496577676626844588240573268701473812127674924007424 - (67682029681889335677290557259385*cos(q2R)*((1917820484151683*cos(q1R))/18014398509481984 + (2579692110316253*sin(q1R))/4503599627370496))/332306998946228968225951765070086144 + (9007199067919185*sin(q2R)*((2579692110316253*cos(q1R))/4503599627370496 - (1917820484151683*sin(q1R))/18014398509481984))/9007199254740992 + 206672498930123057048696703425560088887371380901/6129982163463555433433388108601236734474956488734408704))/9007199254740992))/16225927682921336339157801028812800 - (48638874966763599*sin(q6R)*((9007199067919185*((7514214926474921*cos(q4R))/36893488147419103232 + (4503599440548691*sin(q4R))/4503599627370496)*(cos(q3R)*(cos(q2R)*((2579692110316253*cos(q1R))/4503599627370496 - (1917820484151683*sin(q1R))/18014398509481984) - (32968958366167862000829996477285*sin(q2R))/40564819207303340847894502572032 + (7514214926474921*sin(q2R)*((1917820484151683*cos(q1R))/18014398509481984 + (2579692110316253*sin(q1R))/4503599627370496))/36893488147419103232) - (9007199067919185*sin(q3R)*((17274190877287359225804725738355*cos(q1R))/162259276829213363391578010288128 + (23235800371559029388956996013805*sin(q1R))/40564819207303340847894502572032 + 27504203825998033884751021716381/166153499473114484112975882535043072))/9007199254740992 + (7514214926474921*sin(q3R)*((32968958366167862000829996477285*cos(q2R))/40564819207303340847894502572032 - (7514214926474921*cos(q2R)*((1917820484151683*cos(q1R))/18014398509481984 + (2579692110316253*sin(q1R))/4503599627370496))/36893488147419103232 + sin(q2R)*((2579692110316253*cos(q1R))/4503599627370496 - (1917820484151683*sin(q1R))/18014398509481984)))/36893488147419103232))/9007199254740992 - (67682029681889335677290557259385*sin(q4R)*((9007199067919185*cos(q3R)*((17274190877287359225804725738355*cos(q1R))/162259276829213363391578010288128 + (23235800371559029388956996013805*sin(q1R))/40564819207303340847894502572032 + 27504203825998033884751021716381/166153499473114484112975882535043072))/9007199254740992 - (7514214926474921*cos(q3R)*((32968958366167862000829996477285*cos(q2R))/40564819207303340847894502572032 - (7514214926474921*cos(q2R)*((1917820484151683*cos(q1R))/18014398509481984 + (2579692110316253*sin(q1R))/4503599627370496))/36893488147419103232 + sin(q2R)*((2579692110316253*cos(q1R))/4503599627370496 - (1917820484151683*sin(q1R))/18014398509481984)))/36893488147419103232 + sin(q3R)*(cos(q2R)*((2579692110316253*cos(q1R))/4503599627370496 - (1917820484151683*sin(q1R))/18014398509481984) - (32968958366167862000829996477285*sin(q2R))/40564819207303340847894502572032 + (7514214926474921*sin(q2R)*((1917820484151683*cos(q1R))/18014398509481984 + (2579692110316253*sin(q1R))/4503599627370496))/36893488147419103232)))/332306998946228968225951765070086144 + (9007199067919185*((9007199067919185*cos(q4R))/9007199254740992 - (234819211581865*sin(q4R))/1152921504606846976)*((129801982932889585091297864435361917839115294955*cos(q1R))/5986310706507378352962293074805895248510699696029696 + (296957971066013582975066703729047659005068212725*cos(q2R))/365375409332725729550921208179070754913983135744 + (174598797980560374072834504815488878557302284405*sin(q1R))/1496577676626844588240573268701473812127674924007424 - (67682029681889335677290557259385*cos(q2R)*((1917820484151683*cos(q1R))/18014398509481984 + (2579692110316253*sin(q1R))/4503599627370496))/332306998946228968225951765070086144 + (9007199067919185*sin(q2R)*((2579692110316253*cos(q1R))/4503599627370496 - (1917820484151683*sin(q1R))/18014398509481984))/9007199254740992 + 206672498930123057048696703425560088887371380901/6129982163463555433433388108601236734474956488734408704))/9007199254740992))/1801439850948198400 - (608651409044468601*cos(q4R)*((9007199067919185*cos(q3R)*((17274190877287359225804725738355*cos(q1R))/162259276829213363391578010288128 + (23235800371559029388956996013805*sin(q1R))/40564819207303340847894502572032 + 27504203825998033884751021716381/166153499473114484112975882535043072))/9007199254740992 - (7514214926474921*cos(q3R)*((32968958366167862000829996477285*cos(q2R))/40564819207303340847894502572032 - (7514214926474921*cos(q2R)*((1917820484151683*cos(q1R))/18014398509481984 + (2579692110316253*sin(q1R))/4503599627370496))/36893488147419103232 + sin(q2R)*((2579692110316253*cos(q1R))/4503599627370496 - (1917820484151683*sin(q1R))/18014398509481984)))/36893488147419103232 + sin(q3R)*(cos(q2R)*((2579692110316253*cos(q1R))/4503599627370496 - (1917820484151683*sin(q1R))/18014398509481984) - (32968958366167862000829996477285*sin(q2R))/40564819207303340847894502572032 + (7514214926474921*sin(q2R)*((1917820484151683*cos(q1R))/18014398509481984 + (2579692110316253*sin(q1R))/4503599627370496))/36893488147419103232)))/73786976294838206464000 - (27*cos(q6R)*(cos(q5R)*((7514214926474921*cos(q4R)*((9007199067919185*cos(q3R)*((17274190877287359225804725738355*cos(q1R))/162259276829213363391578010288128 + (23235800371559029388956996013805*sin(q1R))/40564819207303340847894502572032 + 27504203825998033884751021716381/166153499473114484112975882535043072))/9007199254740992 - (7514214926474921*cos(q3R)*((32968958366167862000829996477285*cos(q2R))/40564819207303340847894502572032 - (7514214926474921*cos(q2R)*((1917820484151683*cos(q1R))/18014398509481984 + (2579692110316253*sin(q1R))/4503599627370496))/36893488147419103232 + sin(q2R)*((2579692110316253*cos(q1R))/4503599627370496 - (1917820484151683*sin(q1R))/18014398509481984)))/36893488147419103232 + sin(q3R)*(cos(q2R)*((2579692110316253*cos(q1R))/4503599627370496 - (1917820484151683*sin(q1R))/18014398509481984) - (32968958366167862000829996477285*sin(q2R))/40564819207303340847894502572032 + (7514214926474921*sin(q2R)*((1917820484151683*cos(q1R))/18014398509481984 + (2579692110316253*sin(q1R))/4503599627370496))/36893488147419103232)))/36893488147419103232 - ((4503599440548691*cos(q4R))/4503599627370496 - (7514214926474921*sin(q4R))/36893488147419103232)*(cos(q3R)*(cos(q2R)*((2579692110316253*cos(q1R))/4503599627370496 - (1917820484151683*sin(q1R))/18014398509481984) - (32968958366167862000829996477285*sin(q2R))/40564819207303340847894502572032 + (7514214926474921*sin(q2R)*((1917820484151683*cos(q1R))/18014398509481984 + (2579692110316253*sin(q1R))/4503599627370496))/36893488147419103232) - (9007199067919185*sin(q3R)*((17274190877287359225804725738355*cos(q1R))/162259276829213363391578010288128 + (23235800371559029388956996013805*sin(q1R))/40564819207303340847894502572032 + 27504203825998033884751021716381/166153499473114484112975882535043072))/9007199254740992 + (7514214926474921*sin(q3R)*((32968958366167862000829996477285*cos(q2R))/40564819207303340847894502572032 - (7514214926474921*cos(q2R)*((1917820484151683*cos(q1R))/18014398509481984 + (2579692110316253*sin(q1R))/4503599627370496))/36893488147419103232 + sin(q2R)*((2579692110316253*cos(q1R))/4503599627370496 - (1917820484151683*sin(q1R))/18014398509481984)))/36893488147419103232) + ((234819211581865*cos(q4R))/1152921504606846976 + (9007199067919185*sin(q4R))/9007199254740992)*((129801982932889585091297864435361917839115294955*cos(q1R))/5986310706507378352962293074805895248510699696029696 + (296957971066013582975066703729047659005068212725*cos(q2R))/365375409332725729550921208179070754913983135744 + (174598797980560374072834504815488878557302284405*sin(q1R))/1496577676626844588240573268701473812127674924007424 - (67682029681889335677290557259385*cos(q2R)*((1917820484151683*cos(q1R))/18014398509481984 + (2579692110316253*sin(q1R))/4503599627370496))/332306998946228968225951765070086144 + (9007199067919185*sin(q2R)*((2579692110316253*cos(q1R))/4503599627370496 - (1917820484151683*sin(q1R))/18014398509481984))/9007199254740992 + 206672498930123057048696703425560088887371380901/6129982163463555433433388108601236734474956488734408704)) - (7514214926474921*sin(q5R)*(((7514214926474921*cos(q4R))/36893488147419103232 + (4503599440548691*sin(q4R))/4503599627370496)*(cos(q3R)*(cos(q2R)*((2579692110316253*cos(q1R))/4503599627370496 - (1917820484151683*sin(q1R))/18014398509481984) - (32968958366167862000829996477285*sin(q2R))/40564819207303340847894502572032 + (7514214926474921*sin(q2R)*((1917820484151683*cos(q1R))/18014398509481984 + (2579692110316253*sin(q1R))/4503599627370496))/36893488147419103232) - (9007199067919185*sin(q3R)*((17274190877287359225804725738355*cos(q1R))/162259276829213363391578010288128 + (23235800371559029388956996013805*sin(q1R))/40564819207303340847894502572032 + 27504203825998033884751021716381/166153499473114484112975882535043072))/9007199254740992 + (7514214926474921*sin(q3R)*((32968958366167862000829996477285*cos(q2R))/40564819207303340847894502572032 - (7514214926474921*cos(q2R)*((1917820484151683*cos(q1R))/18014398509481984 + (2579692110316253*sin(q1R))/4503599627370496))/36893488147419103232 + sin(q2R)*((2579692110316253*cos(q1R))/4503599627370496 - (1917820484151683*sin(q1R))/18014398509481984)))/36893488147419103232) - (7514214926474921*sin(q4R)*((9007199067919185*cos(q3R)*((17274190877287359225804725738355*cos(q1R))/162259276829213363391578010288128 + (23235800371559029388956996013805*sin(q1R))/40564819207303340847894502572032 + 27504203825998033884751021716381/166153499473114484112975882535043072))/9007199254740992 - (7514214926474921*cos(q3R)*((32968958366167862000829996477285*cos(q2R))/40564819207303340847894502572032 - (7514214926474921*cos(q2R)*((1917820484151683*cos(q1R))/18014398509481984 + (2579692110316253*sin(q1R))/4503599627370496))/36893488147419103232 + sin(q2R)*((2579692110316253*cos(q1R))/4503599627370496 - (1917820484151683*sin(q1R))/18014398509481984)))/36893488147419103232 + sin(q3R)*(cos(q2R)*((2579692110316253*cos(q1R))/4503599627370496 - (1917820484151683*sin(q1R))/18014398509481984) - (32968958366167862000829996477285*sin(q2R))/40564819207303340847894502572032 + (7514214926474921*sin(q2R)*((1917820484151683*cos(q1R))/18014398509481984 + (2579692110316253*sin(q1R))/4503599627370496))/36893488147419103232)))/36893488147419103232 + ((9007199067919185*cos(q4R))/9007199254740992 - (234819211581865*sin(q4R))/1152921504606846976)*((129801982932889585091297864435361917839115294955*cos(q1R))/5986310706507378352962293074805895248510699696029696 + (296957971066013582975066703729047659005068212725*cos(q2R))/365375409332725729550921208179070754913983135744 + (174598797980560374072834504815488878557302284405*sin(q1R))/1496577676626844588240573268701473812127674924007424 - (67682029681889335677290557259385*cos(q2R)*((1917820484151683*cos(q1R))/18014398509481984 + (2579692110316253*sin(q1R))/4503599627370496))/332306998946228968225951765070086144 + (9007199067919185*sin(q2R)*((2579692110316253*cos(q1R))/4503599627370496 - (1917820484151683*sin(q1R))/18014398509481984))/9007199254740992 + 206672498930123057048696703425560088887371380901/6129982163463555433433388108601236734474956488734408704)))/36893488147419103232))/1000 - (2436553109258773196144549622003023*cos(q6R)*((7514214926474921*cos(q5R)*(((7514214926474921*cos(q4R))/36893488147419103232 + (4503599440548691*sin(q4R))/4503599627370496)*(cos(q3R)*(cos(q2R)*((2579692110316253*cos(q1R))/4503599627370496 - (1917820484151683*sin(q1R))/18014398509481984) - (32968958366167862000829996477285*sin(q2R))/40564819207303340847894502572032 + (7514214926474921*sin(q2R)*((1917820484151683*cos(q1R))/18014398509481984 + (2579692110316253*sin(q1R))/4503599627370496))/36893488147419103232) - (9007199067919185*sin(q3R)*((17274190877287359225804725738355*cos(q1R))/162259276829213363391578010288128 + (23235800371559029388956996013805*sin(q1R))/40564819207303340847894502572032 + 27504203825998033884751021716381/166153499473114484112975882535043072))/9007199254740992 + (7514214926474921*sin(q3R)*((32968958366167862000829996477285*cos(q2R))/40564819207303340847894502572032 - (7514214926474921*cos(q2R)*((1917820484151683*cos(q1R))/18014398509481984 + (2579692110316253*sin(q1R))/4503599627370496))/36893488147419103232 + sin(q2R)*((2579692110316253*cos(q1R))/4503599627370496 - (1917820484151683*sin(q1R))/18014398509481984)))/36893488147419103232) - (7514214926474921*sin(q4R)*((9007199067919185*cos(q3R)*((17274190877287359225804725738355*cos(q1R))/162259276829213363391578010288128 + (23235800371559029388956996013805*sin(q1R))/40564819207303340847894502572032 + 27504203825998033884751021716381/166153499473114484112975882535043072))/9007199254740992 - (7514214926474921*cos(q3R)*((32968958366167862000829996477285*cos(q2R))/40564819207303340847894502572032 - (7514214926474921*cos(q2R)*((1917820484151683*cos(q1R))/18014398509481984 + (2579692110316253*sin(q1R))/4503599627370496))/36893488147419103232 + sin(q2R)*((2579692110316253*cos(q1R))/4503599627370496 - (1917820484151683*sin(q1R))/18014398509481984)))/36893488147419103232 + sin(q3R)*(cos(q2R)*((2579692110316253*cos(q1R))/4503599627370496 - (1917820484151683*sin(q1R))/18014398509481984) - (32968958366167862000829996477285*sin(q2R))/40564819207303340847894502572032 + (7514214926474921*sin(q2R)*((1917820484151683*cos(q1R))/18014398509481984 + (2579692110316253*sin(q1R))/4503599627370496))/36893488147419103232)))/36893488147419103232 + ((9007199067919185*cos(q4R))/9007199254740992 - (234819211581865*sin(q4R))/1152921504606846976)*((129801982932889585091297864435361917839115294955*cos(q1R))/5986310706507378352962293074805895248510699696029696 + (296957971066013582975066703729047659005068212725*cos(q2R))/365375409332725729550921208179070754913983135744 + (174598797980560374072834504815488878557302284405*sin(q1R))/1496577676626844588240573268701473812127674924007424 - (67682029681889335677290557259385*cos(q2R)*((1917820484151683*cos(q1R))/18014398509481984 + (2579692110316253*sin(q1R))/4503599627370496))/332306998946228968225951765070086144 + (9007199067919185*sin(q2R)*((2579692110316253*cos(q1R))/4503599627370496 - (1917820484151683*sin(q1R))/18014398509481984))/9007199254740992 + 206672498930123057048696703425560088887371380901/6129982163463555433433388108601236734474956488734408704)))/36893488147419103232 + sin(q5R)*((7514214926474921*cos(q4R)*((9007199067919185*cos(q3R)*((17274190877287359225804725738355*cos(q1R))/162259276829213363391578010288128 + (23235800371559029388956996013805*sin(q1R))/40564819207303340847894502572032 + 27504203825998033884751021716381/166153499473114484112975882535043072))/9007199254740992 - (7514214926474921*cos(q3R)*((32968958366167862000829996477285*cos(q2R))/40564819207303340847894502572032 - (7514214926474921*cos(q2R)*((1917820484151683*cos(q1R))/18014398509481984 + (2579692110316253*sin(q1R))/4503599627370496))/36893488147419103232 + sin(q2R)*((2579692110316253*cos(q1R))/4503599627370496 - (1917820484151683*sin(q1R))/18014398509481984)))/36893488147419103232 + sin(q3R)*(cos(q2R)*((2579692110316253*cos(q1R))/4503599627370496 - (1917820484151683*sin(q1R))/18014398509481984) - (32968958366167862000829996477285*sin(q2R))/40564819207303340847894502572032 + (7514214926474921*sin(q2R)*((1917820484151683*cos(q1R))/18014398509481984 + (2579692110316253*sin(q1R))/4503599627370496))/36893488147419103232)))/36893488147419103232 - ((4503599440548691*cos(q4R))/4503599627370496 - (7514214926474921*sin(q4R))/36893488147419103232)*(cos(q3R)*(cos(q2R)*((2579692110316253*cos(q1R))/4503599627370496 - (1917820484151683*sin(q1R))/18014398509481984) - (32968958366167862000829996477285*sin(q2R))/40564819207303340847894502572032 + (7514214926474921*sin(q2R)*((1917820484151683*cos(q1R))/18014398509481984 + (2579692110316253*sin(q1R))/4503599627370496))/36893488147419103232) - (9007199067919185*sin(q3R)*((17274190877287359225804725738355*cos(q1R))/162259276829213363391578010288128 + (23235800371559029388956996013805*sin(q1R))/40564819207303340847894502572032 + 27504203825998033884751021716381/166153499473114484112975882535043072))/9007199254740992 + (7514214926474921*sin(q3R)*((32968958366167862000829996477285*cos(q2R))/40564819207303340847894502572032 - (7514214926474921*cos(q2R)*((1917820484151683*cos(q1R))/18014398509481984 + (2579692110316253*sin(q1R))/4503599627370496))/36893488147419103232 + sin(q2R)*((2579692110316253*cos(q1R))/4503599627370496 - (1917820484151683*sin(q1R))/18014398509481984)))/36893488147419103232) + ((234819211581865*cos(q4R))/1152921504606846976 + (9007199067919185*sin(q4R))/9007199254740992)*((129801982932889585091297864435361917839115294955*cos(q1R))/5986310706507378352962293074805895248510699696029696 + (296957971066013582975066703729047659005068212725*cos(q2R))/365375409332725729550921208179070754913983135744 + (174598797980560374072834504815488878557302284405*sin(q1R))/1496577676626844588240573268701473812127674924007424 - (67682029681889335677290557259385*cos(q2R)*((1917820484151683*cos(q1R))/18014398509481984 + (2579692110316253*sin(q1R))/4503599627370496))/332306998946228968225951765070086144 + (9007199067919185*sin(q2R)*((2579692110316253*cos(q1R))/4503599627370496 - (1917820484151683*sin(q1R))/18014398509481984))/9007199254740992 + 206672498930123057048696703425560088887371380901/6129982163463555433433388108601236734474956488734408704))))/332306998946228968225951765070086144000 + (27*cos(q5R)*((7514214926474921*cos(q4R)*((9007199067919185*cos(q3R)*((17274190877287359225804725738355*cos(q1R))/162259276829213363391578010288128 + (23235800371559029388956996013805*sin(q1R))/40564819207303340847894502572032 + 27504203825998033884751021716381/166153499473114484112975882535043072))/9007199254740992 - (7514214926474921*cos(q3R)*((32968958366167862000829996477285*cos(q2R))/40564819207303340847894502572032 - (7514214926474921*cos(q2R)*((1917820484151683*cos(q1R))/18014398509481984 + (2579692110316253*sin(q1R))/4503599627370496))/36893488147419103232 + sin(q2R)*((2579692110316253*cos(q1R))/4503599627370496 - (1917820484151683*sin(q1R))/18014398509481984)))/36893488147419103232 + sin(q3R)*(cos(q2R)*((2579692110316253*cos(q1R))/4503599627370496 - (1917820484151683*sin(q1R))/18014398509481984) - (32968958366167862000829996477285*sin(q2R))/40564819207303340847894502572032 + (7514214926474921*sin(q2R)*((1917820484151683*cos(q1R))/18014398509481984 + (2579692110316253*sin(q1R))/4503599627370496))/36893488147419103232)))/36893488147419103232 - ((4503599440548691*cos(q4R))/4503599627370496 - (7514214926474921*sin(q4R))/36893488147419103232)*(cos(q3R)*(cos(q2R)*((2579692110316253*cos(q1R))/4503599627370496 - (1917820484151683*sin(q1R))/18014398509481984) - (32968958366167862000829996477285*sin(q2R))/40564819207303340847894502572032 + (7514214926474921*sin(q2R)*((1917820484151683*cos(q1R))/18014398509481984 + (2579692110316253*sin(q1R))/4503599627370496))/36893488147419103232) - (9007199067919185*sin(q3R)*((17274190877287359225804725738355*cos(q1R))/162259276829213363391578010288128 + (23235800371559029388956996013805*sin(q1R))/40564819207303340847894502572032 + 27504203825998033884751021716381/166153499473114484112975882535043072))/9007199254740992 + (7514214926474921*sin(q3R)*((32968958366167862000829996477285*cos(q2R))/40564819207303340847894502572032 - (7514214926474921*cos(q2R)*((1917820484151683*cos(q1R))/18014398509481984 + (2579692110316253*sin(q1R))/4503599627370496))/36893488147419103232 + sin(q2R)*((2579692110316253*cos(q1R))/4503599627370496 - (1917820484151683*sin(q1R))/18014398509481984)))/36893488147419103232) + ((234819211581865*cos(q4R))/1152921504606846976 + (9007199067919185*sin(q4R))/9007199254740992)*((129801982932889585091297864435361917839115294955*cos(q1R))/5986310706507378352962293074805895248510699696029696 + (296957971066013582975066703729047659005068212725*cos(q2R))/365375409332725729550921208179070754913983135744 + (174598797980560374072834504815488878557302284405*sin(q1R))/1496577676626844588240573268701473812127674924007424 - (67682029681889335677290557259385*cos(q2R)*((1917820484151683*cos(q1R))/18014398509481984 + (2579692110316253*sin(q1R))/4503599627370496))/332306998946228968225951765070086144 + (9007199067919185*sin(q2R)*((2579692110316253*cos(q1R))/4503599627370496 - (1917820484151683*sin(q1R))/18014398509481984))/9007199254740992 + 206672498930123057048696703425560088887371380901/6129982163463555433433388108601236734474956488734408704)))/1000 + (610321541873521657855151997354401418608858870661075444886782706002880706727*sin(q4R)*((9007199067919185*cos(q3R)*((17274190877287359225804725738355*cos(q1R))/162259276829213363391578010288128 + (23235800371559029388956996013805*sin(q1R))/40564819207303340847894502572032 + 27504203825998033884751021716381/166153499473114484112975882535043072))/9007199254740992 - (7514214926474921*cos(q3R)*((32968958366167862000829996477285*cos(q2R))/40564819207303340847894502572032 - (7514214926474921*cos(q2R)*((1917820484151683*cos(q1R))/18014398509481984 + (2579692110316253*sin(q1R))/4503599627370496))/36893488147419103232 + sin(q2R)*((2579692110316253*cos(q1R))/4503599627370496 - (1917820484151683*sin(q1R))/18014398509481984)))/36893488147419103232 + sin(q3R)*(cos(q2R)*((2579692110316253*cos(q1R))/4503599627370496 - (1917820484151683*sin(q1R))/18014398509481984) - (32968958366167862000829996477285*sin(q2R))/40564819207303340847894502572032 + (7514214926474921*sin(q2R)*((1917820484151683*cos(q1R))/18014398509481984 + (2579692110316253*sin(q1R))/4503599627370496))/36893488147419103232)))/11307821214581659709333104004754678501295896940003961331978279688272766566400000 - (81222263116692158804177042061221826384594597321566869716687*((9007199067919185*cos(q4R))/9007199254740992 - (234819211581865*sin(q4R))/1152921504606846976)*((129801982932889585091297864435361917839115294955*cos(q1R))/5986310706507378352962293074805895248510699696029696 + (296957971066013582975066703729047659005068212725*cos(q2R))/365375409332725729550921208179070754913983135744 + (174598797980560374072834504815488878557302284405*sin(q1R))/1496577676626844588240573268701473812127674924007424 - (67682029681889335677290557259385*cos(q2R)*((1917820484151683*cos(q1R))/18014398509481984 + (2579692110316253*sin(q1R))/4503599627370496))/332306998946228968225951765070086144 + (9007199067919185*sin(q2R)*((2579692110316253*cos(q1R))/4503599627370496 - (1917820484151683*sin(q1R))/18014398509481984))/9007199254740992 + 206672498930123057048696703425560088887371380901/6129982163463555433433388108601236734474956488734408704))/306499108173177771671669405430061836723747824436720435200000 - (81*((234819211581865*cos(q4R))/1152921504606846976 + (9007199067919185*sin(q4R))/9007199254740992)*((129801982932889585091297864435361917839115294955*cos(q1R))/5986310706507378352962293074805895248510699696029696 + (296957971066013582975066703729047659005068212725*cos(q2R))/365375409332725729550921208179070754913983135744 + (174598797980560374072834504815488878557302284405*sin(q1R))/1496577676626844588240573268701473812127674924007424 - (67682029681889335677290557259385*cos(q2R)*((1917820484151683*cos(q1R))/18014398509481984 + (2579692110316253*sin(q1R))/4503599627370496))/332306998946228968225951765070086144 + (9007199067919185*sin(q2R)*((2579692110316253*cos(q1R))/4503599627370496 - (1917820484151683*sin(q1R))/18014398509481984))/9007199254740992 + 206672498930123057048696703425560088887371380901/6129982163463555433433388108601236734474956488734408704))/2000 + (324259171862923063*sin(q6R)*(cos(q5R)*((7514214926474921*cos(q4R)*((9007199067919185*cos(q3R)*((17274190877287359225804725738355*cos(q1R))/162259276829213363391578010288128 + (23235800371559029388956996013805*sin(q1R))/40564819207303340847894502572032 + 27504203825998033884751021716381/166153499473114484112975882535043072))/9007199254740992 - (7514214926474921*cos(q3R)*((32968958366167862000829996477285*cos(q2R))/40564819207303340847894502572032 - (7514214926474921*cos(q2R)*((1917820484151683*cos(q1R))/18014398509481984 + (2579692110316253*sin(q1R))/4503599627370496))/36893488147419103232 + sin(q2R)*((2579692110316253*cos(q1R))/4503599627370496 - (1917820484151683*sin(q1R))/18014398509481984)))/36893488147419103232 + sin(q3R)*(cos(q2R)*((2579692110316253*cos(q1R))/4503599627370496 - (1917820484151683*sin(q1R))/18014398509481984) - (32968958366167862000829996477285*sin(q2R))/40564819207303340847894502572032 + (7514214926474921*sin(q2R)*((1917820484151683*cos(q1R))/18014398509481984 + (2579692110316253*sin(q1R))/4503599627370496))/36893488147419103232)))/36893488147419103232 - ((4503599440548691*cos(q4R))/4503599627370496 - (7514214926474921*sin(q4R))/36893488147419103232)*(cos(q3R)*(cos(q2R)*((2579692110316253*cos(q1R))/4503599627370496 - (1917820484151683*sin(q1R))/18014398509481984) - (32968958366167862000829996477285*sin(q2R))/40564819207303340847894502572032 + (7514214926474921*sin(q2R)*((1917820484151683*cos(q1R))/18014398509481984 + (2579692110316253*sin(q1R))/4503599627370496))/36893488147419103232) - (9007199067919185*sin(q3R)*((17274190877287359225804725738355*cos(q1R))/162259276829213363391578010288128 + (23235800371559029388956996013805*sin(q1R))/40564819207303340847894502572032 + 27504203825998033884751021716381/166153499473114484112975882535043072))/9007199254740992 + (7514214926474921*sin(q3R)*((32968958366167862000829996477285*cos(q2R))/40564819207303340847894502572032 - (7514214926474921*cos(q2R)*((1917820484151683*cos(q1R))/18014398509481984 + (2579692110316253*sin(q1R))/4503599627370496))/36893488147419103232 + sin(q2R)*((2579692110316253*cos(q1R))/4503599627370496 - (1917820484151683*sin(q1R))/18014398509481984)))/36893488147419103232) + ((234819211581865*cos(q4R))/1152921504606846976 + (9007199067919185*sin(q4R))/9007199254740992)*((129801982932889585091297864435361917839115294955*cos(q1R))/5986310706507378352962293074805895248510699696029696 + (296957971066013582975066703729047659005068212725*cos(q2R))/365375409332725729550921208179070754913983135744 + (174598797980560374072834504815488878557302284405*sin(q1R))/1496577676626844588240573268701473812127674924007424 - (67682029681889335677290557259385*cos(q2R)*((1917820484151683*cos(q1R))/18014398509481984 + (2579692110316253*sin(q1R))/4503599627370496))/332306998946228968225951765070086144 + (9007199067919185*sin(q2R)*((2579692110316253*cos(q1R))/4503599627370496 - (1917820484151683*sin(q1R))/18014398509481984))/9007199254740992 + 206672498930123057048696703425560088887371380901/6129982163463555433433388108601236734474956488734408704)) - (7514214926474921*sin(q5R)*(((7514214926474921*cos(q4R))/36893488147419103232 + (4503599440548691*sin(q4R))/4503599627370496)*(cos(q3R)*(cos(q2R)*((2579692110316253*cos(q1R))/4503599627370496 - (1917820484151683*sin(q1R))/18014398509481984) - (32968958366167862000829996477285*sin(q2R))/40564819207303340847894502572032 + (7514214926474921*sin(q2R)*((1917820484151683*cos(q1R))/18014398509481984 + (2579692110316253*sin(q1R))/4503599627370496))/36893488147419103232) - (9007199067919185*sin(q3R)*((17274190877287359225804725738355*cos(q1R))/162259276829213363391578010288128 + (23235800371559029388956996013805*sin(q1R))/40564819207303340847894502572032 + 27504203825998033884751021716381/166153499473114484112975882535043072))/9007199254740992 + (7514214926474921*sin(q3R)*((32968958366167862000829996477285*cos(q2R))/40564819207303340847894502572032 - (7514214926474921*cos(q2R)*((1917820484151683*cos(q1R))/18014398509481984 + (2579692110316253*sin(q1R))/4503599627370496))/36893488147419103232 + sin(q2R)*((2579692110316253*cos(q1R))/4503599627370496 - (1917820484151683*sin(q1R))/18014398509481984)))/36893488147419103232) - (7514214926474921*sin(q4R)*((9007199067919185*cos(q3R)*((17274190877287359225804725738355*cos(q1R))/162259276829213363391578010288128 + (23235800371559029388956996013805*sin(q1R))/40564819207303340847894502572032 + 27504203825998033884751021716381/166153499473114484112975882535043072))/9007199254740992 - (7514214926474921*cos(q3R)*((32968958366167862000829996477285*cos(q2R))/40564819207303340847894502572032 - (7514214926474921*cos(q2R)*((1917820484151683*cos(q1R))/18014398509481984 + (2579692110316253*sin(q1R))/4503599627370496))/36893488147419103232 + sin(q2R)*((2579692110316253*cos(q1R))/4503599627370496 - (1917820484151683*sin(q1R))/18014398509481984)))/36893488147419103232 + sin(q3R)*(cos(q2R)*((2579692110316253*cos(q1R))/4503599627370496 - (1917820484151683*sin(q1R))/18014398509481984) - (32968958366167862000829996477285*sin(q2R))/40564819207303340847894502572032 + (7514214926474921*sin(q2R)*((1917820484151683*cos(q1R))/18014398509481984 + (2579692110316253*sin(q1R))/4503599627370496))/36893488147419103232)))/36893488147419103232 + ((9007199067919185*cos(q4R))/9007199254740992 - (234819211581865*sin(q4R))/1152921504606846976)*((129801982932889585091297864435361917839115294955*cos(q1R))/5986310706507378352962293074805895248510699696029696 + (296957971066013582975066703729047659005068212725*cos(q2R))/365375409332725729550921208179070754913983135744 + (174598797980560374072834504815488878557302284405*sin(q1R))/1496577676626844588240573268701473812127674924007424 - (67682029681889335677290557259385*cos(q2R)*((1917820484151683*cos(q1R))/18014398509481984 + (2579692110316253*sin(q1R))/4503599627370496))/332306998946228968225951765070086144 + (9007199067919185*sin(q2R)*((2579692110316253*cos(q1R))/4503599627370496 - (1917820484151683*sin(q1R))/18014398509481984))/9007199254740992 + 206672498930123057048696703425560088887371380901/6129982163463555433433388108601236734474956488734408704)))/36893488147419103232))/9007199254740992000 - (202883803014822867*sin(q6R)*((7514214926474921*cos(q5R)*(((7514214926474921*cos(q4R))/36893488147419103232 + (4503599440548691*sin(q4R))/4503599627370496)*(cos(q3R)*(cos(q2R)*((2579692110316253*cos(q1R))/4503599627370496 - (1917820484151683*sin(q1R))/18014398509481984) - (32968958366167862000829996477285*sin(q2R))/40564819207303340847894502572032 + (7514214926474921*sin(q2R)*((1917820484151683*cos(q1R))/18014398509481984 + (2579692110316253*sin(q1R))/4503599627370496))/36893488147419103232) - (9007199067919185*sin(q3R)*((17274190877287359225804725738355*cos(q1R))/162259276829213363391578010288128 + (23235800371559029388956996013805*sin(q1R))/40564819207303340847894502572032 + 27504203825998033884751021716381/166153499473114484112975882535043072))/9007199254740992 + (7514214926474921*sin(q3R)*((32968958366167862000829996477285*cos(q2R))/40564819207303340847894502572032 - (7514214926474921*cos(q2R)*((1917820484151683*cos(q1R))/18014398509481984 + (2579692110316253*sin(q1R))/4503599627370496))/36893488147419103232 + sin(q2R)*((2579692110316253*cos(q1R))/4503599627370496 - (1917820484151683*sin(q1R))/18014398509481984)))/36893488147419103232) - (7514214926474921*sin(q4R)*((9007199067919185*cos(q3R)*((17274190877287359225804725738355*cos(q1R))/162259276829213363391578010288128 + (23235800371559029388956996013805*sin(q1R))/40564819207303340847894502572032 + 27504203825998033884751021716381/166153499473114484112975882535043072))/9007199254740992 - (7514214926474921*cos(q3R)*((32968958366167862000829996477285*cos(q2R))/40564819207303340847894502572032 - (7514214926474921*cos(q2R)*((1917820484151683*cos(q1R))/18014398509481984 + (2579692110316253*sin(q1R))/4503599627370496))/36893488147419103232 + sin(q2R)*((2579692110316253*cos(q1R))/4503599627370496 - (1917820484151683*sin(q1R))/18014398509481984)))/36893488147419103232 + sin(q3R)*(cos(q2R)*((2579692110316253*cos(q1R))/4503599627370496 - (1917820484151683*sin(q1R))/18014398509481984) - (32968958366167862000829996477285*sin(q2R))/40564819207303340847894502572032 + (7514214926474921*sin(q2R)*((1917820484151683*cos(q1R))/18014398509481984 + (2579692110316253*sin(q1R))/4503599627370496))/36893488147419103232)))/36893488147419103232 + ((9007199067919185*cos(q4R))/9007199254740992 - (234819211581865*sin(q4R))/1152921504606846976)*((129801982932889585091297864435361917839115294955*cos(q1R))/5986310706507378352962293074805895248510699696029696 + (296957971066013582975066703729047659005068212725*cos(q2R))/365375409332725729550921208179070754913983135744 + (174598797980560374072834504815488878557302284405*sin(q1R))/1496577676626844588240573268701473812127674924007424 - (67682029681889335677290557259385*cos(q2R)*((1917820484151683*cos(q1R))/18014398509481984 + (2579692110316253*sin(q1R))/4503599627370496))/332306998946228968225951765070086144 + (9007199067919185*sin(q2R)*((2579692110316253*cos(q1R))/4503599627370496 - (1917820484151683*sin(q1R))/18014398509481984))/9007199254740992 + 206672498930123057048696703425560088887371380901/6129982163463555433433388108601236734474956488734408704)))/36893488147419103232 + sin(q5R)*((7514214926474921*cos(q4R)*((9007199067919185*cos(q3R)*((17274190877287359225804725738355*cos(q1R))/162259276829213363391578010288128 + (23235800371559029388956996013805*sin(q1R))/40564819207303340847894502572032 + 27504203825998033884751021716381/166153499473114484112975882535043072))/9007199254740992 - (7514214926474921*cos(q3R)*((32968958366167862000829996477285*cos(q2R))/40564819207303340847894502572032 - (7514214926474921*cos(q2R)*((1917820484151683*cos(q1R))/18014398509481984 + (2579692110316253*sin(q1R))/4503599627370496))/36893488147419103232 + sin(q2R)*((2579692110316253*cos(q1R))/4503599627370496 - (1917820484151683*sin(q1R))/18014398509481984)))/36893488147419103232 + sin(q3R)*(cos(q2R)*((2579692110316253*cos(q1R))/4503599627370496 - (1917820484151683*sin(q1R))/18014398509481984) - (32968958366167862000829996477285*sin(q2R))/40564819207303340847894502572032 + (7514214926474921*sin(q2R)*((1917820484151683*cos(q1R))/18014398509481984 + (2579692110316253*sin(q1R))/4503599627370496))/36893488147419103232)))/36893488147419103232 - ((4503599440548691*cos(q4R))/4503599627370496 - (7514214926474921*sin(q4R))/36893488147419103232)*(cos(q3R)*(cos(q2R)*((2579692110316253*cos(q1R))/4503599627370496 - (1917820484151683*sin(q1R))/18014398509481984) - (32968958366167862000829996477285*sin(q2R))/40564819207303340847894502572032 + (7514214926474921*sin(q2R)*((1917820484151683*cos(q1R))/18014398509481984 + (2579692110316253*sin(q1R))/4503599627370496))/36893488147419103232) - (9007199067919185*sin(q3R)*((17274190877287359225804725738355*cos(q1R))/162259276829213363391578010288128 + (23235800371559029388956996013805*sin(q1R))/40564819207303340847894502572032 + 27504203825998033884751021716381/166153499473114484112975882535043072))/9007199254740992 + (7514214926474921*sin(q3R)*((32968958366167862000829996477285*cos(q2R))/40564819207303340847894502572032 - (7514214926474921*cos(q2R)*((1917820484151683*cos(q1R))/18014398509481984 + (2579692110316253*sin(q1R))/4503599627370496))/36893488147419103232 + sin(q2R)*((2579692110316253*cos(q1R))/4503599627370496 - (1917820484151683*sin(q1R))/18014398509481984)))/36893488147419103232) + ((234819211581865*cos(q4R))/1152921504606846976 + (9007199067919185*sin(q4R))/9007199254740992)*((129801982932889585091297864435361917839115294955*cos(q1R))/5986310706507378352962293074805895248510699696029696 + (296957971066013582975066703729047659005068212725*cos(q2R))/365375409332725729550921208179070754913983135744 + (174598797980560374072834504815488878557302284405*sin(q1R))/1496577676626844588240573268701473812127674924007424 - (67682029681889335677290557259385*cos(q2R)*((1917820484151683*cos(q1R))/18014398509481984 + (2579692110316253*sin(q1R))/4503599627370496))/332306998946228968225951765070086144 + (9007199067919185*sin(q2R)*((2579692110316253*cos(q1R))/4503599627370496 - (1917820484151683*sin(q1R))/18014398509481984))/9007199254740992 + 206672498930123057048696703425560088887371380901/6129982163463555433433388108601236734474956488734408704))))/36893488147419103232000 + (712008244765680093343103025701132101054572137019*cos(q5R)*(((7514214926474921*cos(q4R))/36893488147419103232 + (4503599440548691*sin(q4R))/4503599627370496)*(cos(q3R)*(cos(q2R)*((2579692110316253*cos(q1R))/4503599627370496 - (1917820484151683*sin(q1R))/18014398509481984) - (32968958366167862000829996477285*sin(q2R))/40564819207303340847894502572032 + (7514214926474921*sin(q2R)*((1917820484151683*cos(q1R))/18014398509481984 + (2579692110316253*sin(q1R))/4503599627370496))/36893488147419103232) - (9007199067919185*sin(q3R)*((17274190877287359225804725738355*cos(q1R))/162259276829213363391578010288128 + (23235800371559029388956996013805*sin(q1R))/40564819207303340847894502572032 + 27504203825998033884751021716381/166153499473114484112975882535043072))/9007199254740992 + (7514214926474921*sin(q3R)*((32968958366167862000829996477285*cos(q2R))/40564819207303340847894502572032 - (7514214926474921*cos(q2R)*((1917820484151683*cos(q1R))/18014398509481984 + (2579692110316253*sin(q1R))/4503599627370496))/36893488147419103232 + sin(q2R)*((2579692110316253*cos(q1R))/4503599627370496 - (1917820484151683*sin(q1R))/18014398509481984)))/36893488147419103232) - (7514214926474921*sin(q4R)*((9007199067919185*cos(q3R)*((17274190877287359225804725738355*cos(q1R))/162259276829213363391578010288128 + (23235800371559029388956996013805*sin(q1R))/40564819207303340847894502572032 + 27504203825998033884751021716381/166153499473114484112975882535043072))/9007199254740992 - (7514214926474921*cos(q3R)*((32968958366167862000829996477285*cos(q2R))/40564819207303340847894502572032 - (7514214926474921*cos(q2R)*((1917820484151683*cos(q1R))/18014398509481984 + (2579692110316253*sin(q1R))/4503599627370496))/36893488147419103232 + sin(q2R)*((2579692110316253*cos(q1R))/4503599627370496 - (1917820484151683*sin(q1R))/18014398509481984)))/36893488147419103232 + sin(q3R)*(cos(q2R)*((2579692110316253*cos(q1R))/4503599627370496 - (1917820484151683*sin(q1R))/18014398509481984) - (32968958366167862000829996477285*sin(q2R))/40564819207303340847894502572032 + (7514214926474921*sin(q2R)*((1917820484151683*cos(q1R))/18014398509481984 + (2579692110316253*sin(q1R))/4503599627370496))/36893488147419103232)))/36893488147419103232 + ((9007199067919185*cos(q4R))/9007199254740992 - (234819211581865*sin(q4R))/1152921504606846976)*((129801982932889585091297864435361917839115294955*cos(q1R))/5986310706507378352962293074805895248510699696029696 + (296957971066013582975066703729047659005068212725*cos(q2R))/365375409332725729550921208179070754913983135744 + (174598797980560374072834504815488878557302284405*sin(q1R))/1496577676626844588240573268701473812127674924007424 - (67682029681889335677290557259385*cos(q2R)*((1917820484151683*cos(q1R))/18014398509481984 + (2579692110316253*sin(q1R))/4503599627370496))/332306998946228968225951765070086144 + (9007199067919185*sin(q2R)*((2579692110316253*cos(q1R))/4503599627370496 - (1917820484151683*sin(q1R))/18014398509481984))/9007199254740992 + 206672498930123057048696703425560088887371380901/6129982163463555433433388108601236734474956488734408704)))/2451992865385422173373355243440494693789982595493763481600 + (94754841554645069948206780163139*sin(q5R)*((7514214926474921*cos(q4R)*((9007199067919185*cos(q3R)*((17274190877287359225804725738355*cos(q1R))/162259276829213363391578010288128 + (23235800371559029388956996013805*sin(q1R))/40564819207303340847894502572032 + 27504203825998033884751021716381/166153499473114484112975882535043072))/9007199254740992 - (7514214926474921*cos(q3R)*((32968958366167862000829996477285*cos(q2R))/40564819207303340847894502572032 - (7514214926474921*cos(q2R)*((1917820484151683*cos(q1R))/18014398509481984 + (2579692110316253*sin(q1R))/4503599627370496))/36893488147419103232 + sin(q2R)*((2579692110316253*cos(q1R))/4503599627370496 - (1917820484151683*sin(q1R))/18014398509481984)))/36893488147419103232 + sin(q3R)*(cos(q2R)*((2579692110316253*cos(q1R))/4503599627370496 - (1917820484151683*sin(q1R))/18014398509481984) - (32968958366167862000829996477285*sin(q2R))/40564819207303340847894502572032 + (7514214926474921*sin(q2R)*((1917820484151683*cos(q1R))/18014398509481984 + (2579692110316253*sin(q1R))/4503599627370496))/36893488147419103232)))/36893488147419103232 - ((4503599440548691*cos(q4R))/4503599627370496 - (7514214926474921*sin(q4R))/36893488147419103232)*(cos(q3R)*(cos(q2R)*((2579692110316253*cos(q1R))/4503599627370496 - (1917820484151683*sin(q1R))/18014398509481984) - (32968958366167862000829996477285*sin(q2R))/40564819207303340847894502572032 + (7514214926474921*sin(q2R)*((1917820484151683*cos(q1R))/18014398509481984 + (2579692110316253*sin(q1R))/4503599627370496))/36893488147419103232) - (9007199067919185*sin(q3R)*((17274190877287359225804725738355*cos(q1R))/162259276829213363391578010288128 + (23235800371559029388956996013805*sin(q1R))/40564819207303340847894502572032 + 27504203825998033884751021716381/166153499473114484112975882535043072))/9007199254740992 + (7514214926474921*sin(q3R)*((32968958366167862000829996477285*cos(q2R))/40564819207303340847894502572032 - (7514214926474921*cos(q2R)*((1917820484151683*cos(q1R))/18014398509481984 + (2579692110316253*sin(q1R))/4503599627370496))/36893488147419103232 + sin(q2R)*((2579692110316253*cos(q1R))/4503599627370496 - (1917820484151683*sin(q1R))/18014398509481984)))/36893488147419103232) + ((234819211581865*cos(q4R))/1152921504606846976 + (9007199067919185*sin(q4R))/9007199254740992)*((129801982932889585091297864435361917839115294955*cos(q1R))/5986310706507378352962293074805895248510699696029696 + (296957971066013582975066703729047659005068212725*cos(q2R))/365375409332725729550921208179070754913983135744 + (174598797980560374072834504815488878557302284405*sin(q1R))/1496577676626844588240573268701473812127674924007424 - (67682029681889335677290557259385*cos(q2R)*((1917820484151683*cos(q1R))/18014398509481984 + (2579692110316253*sin(q1R))/4503599627370496))/332306998946228968225951765070086144 + (9007199067919185*sin(q2R)*((2579692110316253*cos(q1R))/4503599627370496 - (1917820484151683*sin(q1R))/18014398509481984))/9007199254740992 + 206672498930123057048696703425560088887371380901/6129982163463555433433388108601236734474956488734408704)))/66461399789245793645190353014017228800 - (202883803014822867*sin(q5R)*(((7514214926474921*cos(q4R))/36893488147419103232 + (4503599440548691*sin(q4R))/4503599627370496)*(cos(q3R)*(cos(q2R)*((2579692110316253*cos(q1R))/4503599627370496 - (1917820484151683*sin(q1R))/18014398509481984) - (32968958366167862000829996477285*sin(q2R))/40564819207303340847894502572032 + (7514214926474921*sin(q2R)*((1917820484151683*cos(q1R))/18014398509481984 + (2579692110316253*sin(q1R))/4503599627370496))/36893488147419103232) - (9007199067919185*sin(q3R)*((17274190877287359225804725738355*cos(q1R))/162259276829213363391578010288128 + (23235800371559029388956996013805*sin(q1R))/40564819207303340847894502572032 + 27504203825998033884751021716381/166153499473114484112975882535043072))/9007199254740992 + (7514214926474921*sin(q3R)*((32968958366167862000829996477285*cos(q2R))/40564819207303340847894502572032 - (7514214926474921*cos(q2R)*((1917820484151683*cos(q1R))/18014398509481984 + (2579692110316253*sin(q1R))/4503599627370496))/36893488147419103232 + sin(q2R)*((2579692110316253*cos(q1R))/4503599627370496 - (1917820484151683*sin(q1R))/18014398509481984)))/36893488147419103232) - (7514214926474921*sin(q4R)*((9007199067919185*cos(q3R)*((17274190877287359225804725738355*cos(q1R))/162259276829213363391578010288128 + (23235800371559029388956996013805*sin(q1R))/40564819207303340847894502572032 + 27504203825998033884751021716381/166153499473114484112975882535043072))/9007199254740992 - (7514214926474921*cos(q3R)*((32968958366167862000829996477285*cos(q2R))/40564819207303340847894502572032 - (7514214926474921*cos(q2R)*((1917820484151683*cos(q1R))/18014398509481984 + (2579692110316253*sin(q1R))/4503599627370496))/36893488147419103232 + sin(q2R)*((2579692110316253*cos(q1R))/4503599627370496 - (1917820484151683*sin(q1R))/18014398509481984)))/36893488147419103232 + sin(q3R)*(cos(q2R)*((2579692110316253*cos(q1R))/4503599627370496 - (1917820484151683*sin(q1R))/18014398509481984) - (32968958366167862000829996477285*sin(q2R))/40564819207303340847894502572032 + (7514214926474921*sin(q2R)*((1917820484151683*cos(q1R))/18014398509481984 + (2579692110316253*sin(q1R))/4503599627370496))/36893488147419103232)))/36893488147419103232 + ((9007199067919185*cos(q4R))/9007199254740992 - (234819211581865*sin(q4R))/1152921504606846976)*((129801982932889585091297864435361917839115294955*cos(q1R))/5986310706507378352962293074805895248510699696029696 + (296957971066013582975066703729047659005068212725*cos(q2R))/365375409332725729550921208179070754913983135744 + (174598797980560374072834504815488878557302284405*sin(q1R))/1496577676626844588240573268701473812127674924007424 - (67682029681889335677290557259385*cos(q2R)*((1917820484151683*cos(q1R))/18014398509481984 + (2579692110316253*sin(q1R))/4503599627370496))/332306998946228968225951765070086144 + (9007199067919185*sin(q2R)*((2579692110316253*cos(q1R))/4503599627370496 - (1917820484151683*sin(q1R))/18014398509481984))/9007199254740992 + 206672498930123057048696703425560088887371380901/6129982163463555433433388108601236734474956488734408704)))/36893488147419103232000, (202883803014822867*sin(q6R)*(cos(q5R)*(((7514214926474921*cos(q4R))/36893488147419103232 + (4503599440548691*sin(q4R))/4503599627370496)*(cos(q3R)*(cos(q2R)*((2579692110316253*cos(q1R))/4503599627370496 - (1917820484151683*sin(q1R))/18014398509481984) - (32968958366167862000829996477285*sin(q2R))/40564819207303340847894502572032 + (7514214926474921*sin(q2R)*((1917820484151683*cos(q1R))/18014398509481984 + (2579692110316253*sin(q1R))/4503599627370496))/36893488147419103232) - (9007199067919185*sin(q3R)*((17274190877287359225804725738355*cos(q1R))/162259276829213363391578010288128 + (23235800371559029388956996013805*sin(q1R))/40564819207303340847894502572032 + 27504203825998033884751021716381/166153499473114484112975882535043072))/9007199254740992 + (7514214926474921*sin(q3R)*((32968958366167862000829996477285*cos(q2R))/40564819207303340847894502572032 - (7514214926474921*cos(q2R)*((1917820484151683*cos(q1R))/18014398509481984 + (2579692110316253*sin(q1R))/4503599627370496))/36893488147419103232 + sin(q2R)*((2579692110316253*cos(q1R))/4503599627370496 - (1917820484151683*sin(q1R))/18014398509481984)))/36893488147419103232) - (7514214926474921*sin(q4R)*((9007199067919185*cos(q3R)*((17274190877287359225804725738355*cos(q1R))/162259276829213363391578010288128 + (23235800371559029388956996013805*sin(q1R))/40564819207303340847894502572032 + 27504203825998033884751021716381/166153499473114484112975882535043072))/9007199254740992 - (7514214926474921*cos(q3R)*((32968958366167862000829996477285*cos(q2R))/40564819207303340847894502572032 - (7514214926474921*cos(q2R)*((1917820484151683*cos(q1R))/18014398509481984 + (2579692110316253*sin(q1R))/4503599627370496))/36893488147419103232 + sin(q2R)*((2579692110316253*cos(q1R))/4503599627370496 - (1917820484151683*sin(q1R))/18014398509481984)))/36893488147419103232 + sin(q3R)*(cos(q2R)*((2579692110316253*cos(q1R))/4503599627370496 - (1917820484151683*sin(q1R))/18014398509481984) - (32968958366167862000829996477285*sin(q2R))/40564819207303340847894502572032 + (7514214926474921*sin(q2R)*((1917820484151683*cos(q1R))/18014398509481984 + (2579692110316253*sin(q1R))/4503599627370496))/36893488147419103232)))/36893488147419103232 + ((9007199067919185*cos(q4R))/9007199254740992 - (234819211581865*sin(q4R))/1152921504606846976)*((129801982932889585091297864435361917839115294955*cos(q1R))/5986310706507378352962293074805895248510699696029696 + (296957971066013582975066703729047659005068212725*cos(q2R))/365375409332725729550921208179070754913983135744 + (174598797980560374072834504815488878557302284405*sin(q1R))/1496577676626844588240573268701473812127674924007424 - (67682029681889335677290557259385*cos(q2R)*((1917820484151683*cos(q1R))/18014398509481984 + (2579692110316253*sin(q1R))/4503599627370496))/332306998946228968225951765070086144 + (9007199067919185*sin(q2R)*((2579692110316253*cos(q1R))/4503599627370496 - (1917820484151683*sin(q1R))/18014398509481984))/9007199254740992 + 206672498930123057048696703425560088887371380901/6129982163463555433433388108601236734474956488734408704)) - (9007199067919185*sin(q5R)*((203422408166946418981152780445187297537016008229516441756292125*cos(q1R))/226156424291633194186662080095093570025917938800079226639565593765455331328 + (465385075279251052437186083221547446448384963368966483726351875*cos(q2R))/13803492693581127574869511724554050904902217944340773110325048447598592 + (273626851807209941619219010639387076236787289365779842797695875*sin(q1R))/56539106072908298546665520023773392506479484700019806659891398441363832832 - (81129635049124235038645691064225*cos(q3R)*((17274190877287359225804725738355*cos(q1R))/162259276829213363391578010288128 + (23235800371559029388956996013805*sin(q1R))/40564819207303340847894502572032 + 27504203825998033884751021716381/166153499473114484112975882535043072))/81129638414606681695789005144064 + (2115063383689692319117831580025*sin(q3R)*((17274190877287359225804725738355*cos(q1R))/162259276829213363391578010288128 + (23235800371559029388956996013805*sin(q1R))/40564819207303340847894502572032 + 27504203825998033884751021716381/166153499473114484112975882535043072))/10384593717069655257060992658440192 + (67682029681889335677290557259385*cos(q3R)*((32968958366167862000829996477285*cos(q2R))/40564819207303340847894502572032 - (7514214926474921*cos(q2R)*((1917820484151683*cos(q1R))/18014398509481984 + (2579692110316253*sin(q1R))/4503599627370496))/36893488147419103232 + sin(q2R)*((2579692110316253*cos(q1R))/4503599627370496 - (1917820484151683*sin(q1R))/18014398509481984)))/332306998946228968225951765070086144 - (234819211581865*cos(q3R)*(cos(q2R)*((2579692110316253*cos(q1R))/4503599627370496 - (1917820484151683*sin(q1R))/18014398509481984) - (32968958366167862000829996477285*sin(q2R))/40564819207303340847894502572032 + (7514214926474921*sin(q2R)*((1917820484151683*cos(q1R))/18014398509481984 + (2579692110316253*sin(q1R))/4503599627370496))/36893488147419103232))/1152921504606846976 - (1764482024691522628700660907665*sin(q3R)*((32968958366167862000829996477285*cos(q2R))/40564819207303340847894502572032 - (7514214926474921*cos(q2R)*((1917820484151683*cos(q1R))/18014398509481984 + (2579692110316253*sin(q1R))/4503599627370496))/36893488147419103232 + sin(q2R)*((2579692110316253*cos(q1R))/4503599627370496 - (1917820484151683*sin(q1R))/18014398509481984)))/42535295865117307932921825928971026432 - (9007199067919185*sin(q3R)*(cos(q2R)*((2579692110316253*cos(q1R))/4503599627370496 - (1917820484151683*sin(q1R))/18014398509481984) - (32968958366167862000829996477285*sin(q2R))/40564819207303340847894502572032 + (7514214926474921*sin(q2R)*((1917820484151683*cos(q1R))/18014398509481984 + (2579692110316253*sin(q1R))/4503599627370496))/36893488147419103232))/9007199254740992 - (106069577339469832923929692356850887620017617375*cos(q2R)*((1917820484151683*cos(q1R))/18014398509481984 + (2579692110316253*sin(q1R))/4503599627370496))/12554203470773361527671578846415332832204710888928069025792 + (14115856197532180673579726082375*sin(q2R)*((2579692110316253*cos(q1R))/4503599627370496 - (1917820484151683*sin(q1R))/18014398509481984))/340282366920938463463374607431768211456 + 323891950525769801103968238055131782751500431270071838086942675/231584178474632390847141970017375815706539969331281128078915168015826259279872))/9007199254740992 + (7514214926474921*sin(q5R)*((7514214926474921*cos(q4R)*((9007199067919185*cos(q3R)*((17274190877287359225804725738355*cos(q1R))/162259276829213363391578010288128 + (23235800371559029388956996013805*sin(q1R))/40564819207303340847894502572032 + 27504203825998033884751021716381/166153499473114484112975882535043072))/9007199254740992 - (7514214926474921*cos(q3R)*((32968958366167862000829996477285*cos(q2R))/40564819207303340847894502572032 - (7514214926474921*cos(q2R)*((1917820484151683*cos(q1R))/18014398509481984 + (2579692110316253*sin(q1R))/4503599627370496))/36893488147419103232 + sin(q2R)*((2579692110316253*cos(q1R))/4503599627370496 - (1917820484151683*sin(q1R))/18014398509481984)))/36893488147419103232 + sin(q3R)*(cos(q2R)*((2579692110316253*cos(q1R))/4503599627370496 - (1917820484151683*sin(q1R))/18014398509481984) - (32968958366167862000829996477285*sin(q2R))/40564819207303340847894502572032 + (7514214926474921*sin(q2R)*((1917820484151683*cos(q1R))/18014398509481984 + (2579692110316253*sin(q1R))/4503599627370496))/36893488147419103232)))/36893488147419103232 - ((4503599440548691*cos(q4R))/4503599627370496 - (7514214926474921*sin(q4R))/36893488147419103232)*(cos(q3R)*(cos(q2R)*((2579692110316253*cos(q1R))/4503599627370496 - (1917820484151683*sin(q1R))/18014398509481984) - (32968958366167862000829996477285*sin(q2R))/40564819207303340847894502572032 + (7514214926474921*sin(q2R)*((1917820484151683*cos(q1R))/18014398509481984 + (2579692110316253*sin(q1R))/4503599627370496))/36893488147419103232) - (9007199067919185*sin(q3R)*((17274190877287359225804725738355*cos(q1R))/162259276829213363391578010288128 + (23235800371559029388956996013805*sin(q1R))/40564819207303340847894502572032 + 27504203825998033884751021716381/166153499473114484112975882535043072))/9007199254740992 + (7514214926474921*sin(q3R)*((32968958366167862000829996477285*cos(q2R))/40564819207303340847894502572032 - (7514214926474921*cos(q2R)*((1917820484151683*cos(q1R))/18014398509481984 + (2579692110316253*sin(q1R))/4503599627370496))/36893488147419103232 + sin(q2R)*((2579692110316253*cos(q1R))/4503599627370496 - (1917820484151683*sin(q1R))/18014398509481984)))/36893488147419103232) + ((234819211581865*cos(q4R))/1152921504606846976 + (9007199067919185*sin(q4R))/9007199254740992)*((129801982932889585091297864435361917839115294955*cos(q1R))/5986310706507378352962293074805895248510699696029696 + (296957971066013582975066703729047659005068212725*cos(q2R))/365375409332725729550921208179070754913983135744 + (174598797980560374072834504815488878557302284405*sin(q1R))/1496577676626844588240573268701473812127674924007424 - (67682029681889335677290557259385*cos(q2R)*((1917820484151683*cos(q1R))/18014398509481984 + (2579692110316253*sin(q1R))/4503599627370496))/332306998946228968225951765070086144 + (9007199067919185*sin(q2R)*((2579692110316253*cos(q1R))/4503599627370496 - (1917820484151683*sin(q1R))/18014398509481984))/9007199254740992 + 206672498930123057048696703425560088887371380901/6129982163463555433433388108601236734474956488734408704)))/36893488147419103232))/36893488147419103232000 + (48638874966763599*cos(q5R)*((203422408166946418981152780445187297537016008229516441756292125*cos(q1R))/226156424291633194186662080095093570025917938800079226639565593765455331328 + (465385075279251052437186083221547446448384963368966483726351875*cos(q2R))/13803492693581127574869511724554050904902217944340773110325048447598592 + (273626851807209941619219010639387076236787289365779842797695875*sin(q1R))/56539106072908298546665520023773392506479484700019806659891398441363832832 - (81129635049124235038645691064225*cos(q3R)*((17274190877287359225804725738355*cos(q1R))/162259276829213363391578010288128 + (23235800371559029388956996013805*sin(q1R))/40564819207303340847894502572032 + 27504203825998033884751021716381/166153499473114484112975882535043072))/81129638414606681695789005144064 + (2115063383689692319117831580025*sin(q3R)*((17274190877287359225804725738355*cos(q1R))/162259276829213363391578010288128 + (23235800371559029388956996013805*sin(q1R))/40564819207303340847894502572032 + 27504203825998033884751021716381/166153499473114484112975882535043072))/10384593717069655257060992658440192 + (67682029681889335677290557259385*cos(q3R)*((32968958366167862000829996477285*cos(q2R))/40564819207303340847894502572032 - (7514214926474921*cos(q2R)*((1917820484151683*cos(q1R))/18014398509481984 + (2579692110316253*sin(q1R))/4503599627370496))/36893488147419103232 + sin(q2R)*((2579692110316253*cos(q1R))/4503599627370496 - (1917820484151683*sin(q1R))/18014398509481984)))/332306998946228968225951765070086144 - (234819211581865*cos(q3R)*(cos(q2R)*((2579692110316253*cos(q1R))/4503599627370496 - (1917820484151683*sin(q1R))/18014398509481984) - (32968958366167862000829996477285*sin(q2R))/40564819207303340847894502572032 + (7514214926474921*sin(q2R)*((1917820484151683*cos(q1R))/18014398509481984 + (2579692110316253*sin(q1R))/4503599627370496))/36893488147419103232))/1152921504606846976 - (1764482024691522628700660907665*sin(q3R)*((32968958366167862000829996477285*cos(q2R))/40564819207303340847894502572032 - (7514214926474921*cos(q2R)*((1917820484151683*cos(q1R))/18014398509481984 + (2579692110316253*sin(q1R))/4503599627370496))/36893488147419103232 + sin(q2R)*((2579692110316253*cos(q1R))/4503599627370496 - (1917820484151683*sin(q1R))/18014398509481984)))/42535295865117307932921825928971026432 - (9007199067919185*sin(q3R)*(cos(q2R)*((2579692110316253*cos(q1R))/4503599627370496 - (1917820484151683*sin(q1R))/18014398509481984) - (32968958366167862000829996477285*sin(q2R))/40564819207303340847894502572032 + (7514214926474921*sin(q2R)*((1917820484151683*cos(q1R))/18014398509481984 + (2579692110316253*sin(q1R))/4503599627370496))/36893488147419103232))/9007199254740992 - (106069577339469832923929692356850887620017617375*cos(q2R)*((1917820484151683*cos(q1R))/18014398509481984 + (2579692110316253*sin(q1R))/4503599627370496))/12554203470773361527671578846415332832204710888928069025792 + (14115856197532180673579726082375*sin(q2R)*((2579692110316253*cos(q1R))/4503599627370496 - (1917820484151683*sin(q1R))/18014398509481984))/340282366920938463463374607431768211456 + 323891950525769801103968238055131782751500431270071838086942675/231584178474632390847141970017375815706539969331281128078915168015826259279872))/1801439850948198400 + (170695144106365826517608855445768431563113584343*sin(q5R)*((203422408166946418981152780445187297537016008229516441756292125*cos(q1R))/226156424291633194186662080095093570025917938800079226639565593765455331328 + (465385075279251052437186083221547446448384963368966483726351875*cos(q2R))/13803492693581127574869511724554050904902217944340773110325048447598592 + (273626851807209941619219010639387076236787289365779842797695875*sin(q1R))/56539106072908298546665520023773392506479484700019806659891398441363832832 - (81129635049124235038645691064225*cos(q3R)*((17274190877287359225804725738355*cos(q1R))/162259276829213363391578010288128 + (23235800371559029388956996013805*sin(q1R))/40564819207303340847894502572032 + 27504203825998033884751021716381/166153499473114484112975882535043072))/81129638414606681695789005144064 + (2115063383689692319117831580025*sin(q3R)*((17274190877287359225804725738355*cos(q1R))/162259276829213363391578010288128 + (23235800371559029388956996013805*sin(q1R))/40564819207303340847894502572032 + 27504203825998033884751021716381/166153499473114484112975882535043072))/10384593717069655257060992658440192 + (67682029681889335677290557259385*cos(q3R)*((32968958366167862000829996477285*cos(q2R))/40564819207303340847894502572032 - (7514214926474921*cos(q2R)*((1917820484151683*cos(q1R))/18014398509481984 + (2579692110316253*sin(q1R))/4503599627370496))/36893488147419103232 + sin(q2R)*((2579692110316253*cos(q1R))/4503599627370496 - (1917820484151683*sin(q1R))/18014398509481984)))/332306998946228968225951765070086144 - (234819211581865*cos(q3R)*(cos(q2R)*((2579692110316253*cos(q1R))/4503599627370496 - (1917820484151683*sin(q1R))/18014398509481984) - (32968958366167862000829996477285*sin(q2R))/40564819207303340847894502572032 + (7514214926474921*sin(q2R)*((1917820484151683*cos(q1R))/18014398509481984 + (2579692110316253*sin(q1R))/4503599627370496))/36893488147419103232))/1152921504606846976 - (1764482024691522628700660907665*sin(q3R)*((32968958366167862000829996477285*cos(q2R))/40564819207303340847894502572032 - (7514214926474921*cos(q2R)*((1917820484151683*cos(q1R))/18014398509481984 + (2579692110316253*sin(q1R))/4503599627370496))/36893488147419103232 + sin(q2R)*((2579692110316253*cos(q1R))/4503599627370496 - (1917820484151683*sin(q1R))/18014398509481984)))/42535295865117307932921825928971026432 - (9007199067919185*sin(q3R)*(cos(q2R)*((2579692110316253*cos(q1R))/4503599627370496 - (1917820484151683*sin(q1R))/18014398509481984) - (32968958366167862000829996477285*sin(q2R))/40564819207303340847894502572032 + (7514214926474921*sin(q2R)*((1917820484151683*cos(q1R))/18014398509481984 + (2579692110316253*sin(q1R))/4503599627370496))/36893488147419103232))/9007199254740992 - (106069577339469832923929692356850887620017617375*cos(q2R)*((1917820484151683*cos(q1R))/18014398509481984 + (2579692110316253*sin(q1R))/4503599627370496))/12554203470773361527671578846415332832204710888928069025792 + (14115856197532180673579726082375*sin(q2R)*((2579692110316253*cos(q1R))/4503599627370496 - (1917820484151683*sin(q1R))/18014398509481984))/340282366920938463463374607431768211456 + 323891950525769801103968238055131782751500431270071838086942675/231584178474632390847141970017375815706539969331281128078915168015826259279872))/119726214130147567059245861496117904970213993920593920 - (202883803014822867*cos(q5R)*((7514214926474921*cos(q4R)*((9007199067919185*cos(q3R)*((17274190877287359225804725738355*cos(q1R))/162259276829213363391578010288128 + (23235800371559029388956996013805*sin(q1R))/40564819207303340847894502572032 + 27504203825998033884751021716381/166153499473114484112975882535043072))/9007199254740992 - (7514214926474921*cos(q3R)*((32968958366167862000829996477285*cos(q2R))/40564819207303340847894502572032 - (7514214926474921*cos(q2R)*((1917820484151683*cos(q1R))/18014398509481984 + (2579692110316253*sin(q1R))/4503599627370496))/36893488147419103232 + sin(q2R)*((2579692110316253*cos(q1R))/4503599627370496 - (1917820484151683*sin(q1R))/18014398509481984)))/36893488147419103232 + sin(q3R)*(cos(q2R)*((2579692110316253*cos(q1R))/4503599627370496 - (1917820484151683*sin(q1R))/18014398509481984) - (32968958366167862000829996477285*sin(q2R))/40564819207303340847894502572032 + (7514214926474921*sin(q2R)*((1917820484151683*cos(q1R))/18014398509481984 + (2579692110316253*sin(q1R))/4503599627370496))/36893488147419103232)))/36893488147419103232 - ((4503599440548691*cos(q4R))/4503599627370496 - (7514214926474921*sin(q4R))/36893488147419103232)*(cos(q3R)*(cos(q2R)*((2579692110316253*cos(q1R))/4503599627370496 - (1917820484151683*sin(q1R))/18014398509481984) - (32968958366167862000829996477285*sin(q2R))/40564819207303340847894502572032 + (7514214926474921*sin(q2R)*((1917820484151683*cos(q1R))/18014398509481984 + (2579692110316253*sin(q1R))/4503599627370496))/36893488147419103232) - (9007199067919185*sin(q3R)*((17274190877287359225804725738355*cos(q1R))/162259276829213363391578010288128 + (23235800371559029388956996013805*sin(q1R))/40564819207303340847894502572032 + 27504203825998033884751021716381/166153499473114484112975882535043072))/9007199254740992 + (7514214926474921*sin(q3R)*((32968958366167862000829996477285*cos(q2R))/40564819207303340847894502572032 - (7514214926474921*cos(q2R)*((1917820484151683*cos(q1R))/18014398509481984 + (2579692110316253*sin(q1R))/4503599627370496))/36893488147419103232 + sin(q2R)*((2579692110316253*cos(q1R))/4503599627370496 - (1917820484151683*sin(q1R))/18014398509481984)))/36893488147419103232) + ((234819211581865*cos(q4R))/1152921504606846976 + (9007199067919185*sin(q4R))/9007199254740992)*((129801982932889585091297864435361917839115294955*cos(q1R))/5986310706507378352962293074805895248510699696029696 + (296957971066013582975066703729047659005068212725*cos(q2R))/365375409332725729550921208179070754913983135744 + (174598797980560374072834504815488878557302284405*sin(q1R))/1496577676626844588240573268701473812127674924007424 - (67682029681889335677290557259385*cos(q2R)*((1917820484151683*cos(q1R))/18014398509481984 + (2579692110316253*sin(q1R))/4503599627370496))/332306998946228968225951765070086144 + (9007199067919185*sin(q2R)*((2579692110316253*cos(q1R))/4503599627370496 - (1917820484151683*sin(q1R))/18014398509481984))/9007199254740992 + 206672498930123057048696703425560088887371380901/6129982163463555433433388108601236734474956488734408704)))/36893488147419103232000 - (94754841554645069948206780163139*cos(q5R)*(((7514214926474921*cos(q4R))/36893488147419103232 + (4503599440548691*sin(q4R))/4503599627370496)*(cos(q3R)*(cos(q2R)*((2579692110316253*cos(q1R))/4503599627370496 - (1917820484151683*sin(q1R))/18014398509481984) - (32968958366167862000829996477285*sin(q2R))/40564819207303340847894502572032 + (7514214926474921*sin(q2R)*((1917820484151683*cos(q1R))/18014398509481984 + (2579692110316253*sin(q1R))/4503599627370496))/36893488147419103232) - (9007199067919185*sin(q3R)*((17274190877287359225804725738355*cos(q1R))/162259276829213363391578010288128 + (23235800371559029388956996013805*sin(q1R))/40564819207303340847894502572032 + 27504203825998033884751021716381/166153499473114484112975882535043072))/9007199254740992 + (7514214926474921*sin(q3R)*((32968958366167862000829996477285*cos(q2R))/40564819207303340847894502572032 - (7514214926474921*cos(q2R)*((1917820484151683*cos(q1R))/18014398509481984 + (2579692110316253*sin(q1R))/4503599627370496))/36893488147419103232 + sin(q2R)*((2579692110316253*cos(q1R))/4503599627370496 - (1917820484151683*sin(q1R))/18014398509481984)))/36893488147419103232) - (7514214926474921*sin(q4R)*((9007199067919185*cos(q3R)*((17274190877287359225804725738355*cos(q1R))/162259276829213363391578010288128 + (23235800371559029388956996013805*sin(q1R))/40564819207303340847894502572032 + 27504203825998033884751021716381/166153499473114484112975882535043072))/9007199254740992 - (7514214926474921*cos(q3R)*((32968958366167862000829996477285*cos(q2R))/40564819207303340847894502572032 - (7514214926474921*cos(q2R)*((1917820484151683*cos(q1R))/18014398509481984 + (2579692110316253*sin(q1R))/4503599627370496))/36893488147419103232 + sin(q2R)*((2579692110316253*cos(q1R))/4503599627370496 - (1917820484151683*sin(q1R))/18014398509481984)))/36893488147419103232 + sin(q3R)*(cos(q2R)*((2579692110316253*cos(q1R))/4503599627370496 - (1917820484151683*sin(q1R))/18014398509481984) - (32968958366167862000829996477285*sin(q2R))/40564819207303340847894502572032 + (7514214926474921*sin(q2R)*((1917820484151683*cos(q1R))/18014398509481984 + (2579692110316253*sin(q1R))/4503599627370496))/36893488147419103232)))/36893488147419103232 + ((9007199067919185*cos(q4R))/9007199254740992 - (234819211581865*sin(q4R))/1152921504606846976)*((129801982932889585091297864435361917839115294955*cos(q1R))/5986310706507378352962293074805895248510699696029696 + (296957971066013582975066703729047659005068212725*cos(q2R))/365375409332725729550921208179070754913983135744 + (174598797980560374072834504815488878557302284405*sin(q1R))/1496577676626844588240573268701473812127674924007424 - (67682029681889335677290557259385*cos(q2R)*((1917820484151683*cos(q1R))/18014398509481984 + (2579692110316253*sin(q1R))/4503599627370496))/332306998946228968225951765070086144 + (9007199067919185*sin(q2R)*((2579692110316253*cos(q1R))/4503599627370496 - (1917820484151683*sin(q1R))/18014398509481984))/9007199254740992 + 206672498930123057048696703425560088887371380901/6129982163463555433433388108601236734474956488734408704)))/66461399789245793645190353014017228800 - (712008244765680093343103025701132101054572137019*sin(q5R)*((7514214926474921*cos(q4R)*((9007199067919185*cos(q3R)*((17274190877287359225804725738355*cos(q1R))/162259276829213363391578010288128 + (23235800371559029388956996013805*sin(q1R))/40564819207303340847894502572032 + 27504203825998033884751021716381/166153499473114484112975882535043072))/9007199254740992 - (7514214926474921*cos(q3R)*((32968958366167862000829996477285*cos(q2R))/40564819207303340847894502572032 - (7514214926474921*cos(q2R)*((1917820484151683*cos(q1R))/18014398509481984 + (2579692110316253*sin(q1R))/4503599627370496))/36893488147419103232 + sin(q2R)*((2579692110316253*cos(q1R))/4503599627370496 - (1917820484151683*sin(q1R))/18014398509481984)))/36893488147419103232 + sin(q3R)*(cos(q2R)*((2579692110316253*cos(q1R))/4503599627370496 - (1917820484151683*sin(q1R))/18014398509481984) - (32968958366167862000829996477285*sin(q2R))/40564819207303340847894502572032 + (7514214926474921*sin(q2R)*((1917820484151683*cos(q1R))/18014398509481984 + (2579692110316253*sin(q1R))/4503599627370496))/36893488147419103232)))/36893488147419103232 - ((4503599440548691*cos(q4R))/4503599627370496 - (7514214926474921*sin(q4R))/36893488147419103232)*(cos(q3R)*(cos(q2R)*((2579692110316253*cos(q1R))/4503599627370496 - (1917820484151683*sin(q1R))/18014398509481984) - (32968958366167862000829996477285*sin(q2R))/40564819207303340847894502572032 + (7514214926474921*sin(q2R)*((1917820484151683*cos(q1R))/18014398509481984 + (2579692110316253*sin(q1R))/4503599627370496))/36893488147419103232) - (9007199067919185*sin(q3R)*((17274190877287359225804725738355*cos(q1R))/162259276829213363391578010288128 + (23235800371559029388956996013805*sin(q1R))/40564819207303340847894502572032 + 27504203825998033884751021716381/166153499473114484112975882535043072))/9007199254740992 + (7514214926474921*sin(q3R)*((32968958366167862000829996477285*cos(q2R))/40564819207303340847894502572032 - (7514214926474921*cos(q2R)*((1917820484151683*cos(q1R))/18014398509481984 + (2579692110316253*sin(q1R))/4503599627370496))/36893488147419103232 + sin(q2R)*((2579692110316253*cos(q1R))/4503599627370496 - (1917820484151683*sin(q1R))/18014398509481984)))/36893488147419103232) + ((234819211581865*cos(q4R))/1152921504606846976 + (9007199067919185*sin(q4R))/9007199254740992)*((129801982932889585091297864435361917839115294955*cos(q1R))/5986310706507378352962293074805895248510699696029696 + (296957971066013582975066703729047659005068212725*cos(q2R))/365375409332725729550921208179070754913983135744 + (174598797980560374072834504815488878557302284405*sin(q1R))/1496577676626844588240573268701473812127674924007424 - (67682029681889335677290557259385*cos(q2R)*((1917820484151683*cos(q1R))/18014398509481984 + (2579692110316253*sin(q1R))/4503599627370496))/332306998946228968225951765070086144 + (9007199067919185*sin(q2R)*((2579692110316253*cos(q1R))/4503599627370496 - (1917820484151683*sin(q1R))/18014398509481984))/9007199254740992 + 206672498930123057048696703425560088887371380901/6129982163463555433433388108601236734474956488734408704)))/2451992865385422173373355243440494693789982595493763481600 + (27*sin(q5R)*(((7514214926474921*cos(q4R))/36893488147419103232 + (4503599440548691*sin(q4R))/4503599627370496)*(cos(q3R)*(cos(q2R)*((2579692110316253*cos(q1R))/4503599627370496 - (1917820484151683*sin(q1R))/18014398509481984) - (32968958366167862000829996477285*sin(q2R))/40564819207303340847894502572032 + (7514214926474921*sin(q2R)*((1917820484151683*cos(q1R))/18014398509481984 + (2579692110316253*sin(q1R))/4503599627370496))/36893488147419103232) - (9007199067919185*sin(q3R)*((17274190877287359225804725738355*cos(q1R))/162259276829213363391578010288128 + (23235800371559029388956996013805*sin(q1R))/40564819207303340847894502572032 + 27504203825998033884751021716381/166153499473114484112975882535043072))/9007199254740992 + (7514214926474921*sin(q3R)*((32968958366167862000829996477285*cos(q2R))/40564819207303340847894502572032 - (7514214926474921*cos(q2R)*((1917820484151683*cos(q1R))/18014398509481984 + (2579692110316253*sin(q1R))/4503599627370496))/36893488147419103232 + sin(q2R)*((2579692110316253*cos(q1R))/4503599627370496 - (1917820484151683*sin(q1R))/18014398509481984)))/36893488147419103232) - (7514214926474921*sin(q4R)*((9007199067919185*cos(q3R)*((17274190877287359225804725738355*cos(q1R))/162259276829213363391578010288128 + (23235800371559029388956996013805*sin(q1R))/40564819207303340847894502572032 + 27504203825998033884751021716381/166153499473114484112975882535043072))/9007199254740992 - (7514214926474921*cos(q3R)*((32968958366167862000829996477285*cos(q2R))/40564819207303340847894502572032 - (7514214926474921*cos(q2R)*((1917820484151683*cos(q1R))/18014398509481984 + (2579692110316253*sin(q1R))/4503599627370496))/36893488147419103232 + sin(q2R)*((2579692110316253*cos(q1R))/4503599627370496 - (1917820484151683*sin(q1R))/18014398509481984)))/36893488147419103232 + sin(q3R)*(cos(q2R)*((2579692110316253*cos(q1R))/4503599627370496 - (1917820484151683*sin(q1R))/18014398509481984) - (32968958366167862000829996477285*sin(q2R))/40564819207303340847894502572032 + (7514214926474921*sin(q2R)*((1917820484151683*cos(q1R))/18014398509481984 + (2579692110316253*sin(q1R))/4503599627370496))/36893488147419103232)))/36893488147419103232 + ((9007199067919185*cos(q4R))/9007199254740992 - (234819211581865*sin(q4R))/1152921504606846976)*((129801982932889585091297864435361917839115294955*cos(q1R))/5986310706507378352962293074805895248510699696029696 + (296957971066013582975066703729047659005068212725*cos(q2R))/365375409332725729550921208179070754913983135744 + (174598797980560374072834504815488878557302284405*sin(q1R))/1496577676626844588240573268701473812127674924007424 - (67682029681889335677290557259385*cos(q2R)*((1917820484151683*cos(q1R))/18014398509481984 + (2579692110316253*sin(q1R))/4503599627370496))/332306998946228968225951765070086144 + (9007199067919185*sin(q2R)*((2579692110316253*cos(q1R))/4503599627370496 - (1917820484151683*sin(q1R))/18014398509481984))/9007199254740992 + 206672498930123057048696703425560088887371380901/6129982163463555433433388108601236734474956488734408704)))/1000 - (27*cos(q6R)*((9007199067919185*cos(q5R)*((203422408166946418981152780445187297537016008229516441756292125*cos(q1R))/226156424291633194186662080095093570025917938800079226639565593765455331328 + (465385075279251052437186083221547446448384963368966483726351875*cos(q2R))/13803492693581127574869511724554050904902217944340773110325048447598592 + (273626851807209941619219010639387076236787289365779842797695875*sin(q1R))/56539106072908298546665520023773392506479484700019806659891398441363832832 - (81129635049124235038645691064225*cos(q3R)*((17274190877287359225804725738355*cos(q1R))/162259276829213363391578010288128 + (23235800371559029388956996013805*sin(q1R))/40564819207303340847894502572032 + 27504203825998033884751021716381/166153499473114484112975882535043072))/81129638414606681695789005144064 + (2115063383689692319117831580025*sin(q3R)*((17274190877287359225804725738355*cos(q1R))/162259276829213363391578010288128 + (23235800371559029388956996013805*sin(q1R))/40564819207303340847894502572032 + 27504203825998033884751021716381/166153499473114484112975882535043072))/10384593717069655257060992658440192 + (67682029681889335677290557259385*cos(q3R)*((32968958366167862000829996477285*cos(q2R))/40564819207303340847894502572032 - (7514214926474921*cos(q2R)*((1917820484151683*cos(q1R))/18014398509481984 + (2579692110316253*sin(q1R))/4503599627370496))/36893488147419103232 + sin(q2R)*((2579692110316253*cos(q1R))/4503599627370496 - (1917820484151683*sin(q1R))/18014398509481984)))/332306998946228968225951765070086144 - (234819211581865*cos(q3R)*(cos(q2R)*((2579692110316253*cos(q1R))/4503599627370496 - (1917820484151683*sin(q1R))/18014398509481984) - (32968958366167862000829996477285*sin(q2R))/40564819207303340847894502572032 + (7514214926474921*sin(q2R)*((1917820484151683*cos(q1R))/18014398509481984 + (2579692110316253*sin(q1R))/4503599627370496))/36893488147419103232))/1152921504606846976 - (1764482024691522628700660907665*sin(q3R)*((32968958366167862000829996477285*cos(q2R))/40564819207303340847894502572032 - (7514214926474921*cos(q2R)*((1917820484151683*cos(q1R))/18014398509481984 + (2579692110316253*sin(q1R))/4503599627370496))/36893488147419103232 + sin(q2R)*((2579692110316253*cos(q1R))/4503599627370496 - (1917820484151683*sin(q1R))/18014398509481984)))/42535295865117307932921825928971026432 - (9007199067919185*sin(q3R)*(cos(q2R)*((2579692110316253*cos(q1R))/4503599627370496 - (1917820484151683*sin(q1R))/18014398509481984) - (32968958366167862000829996477285*sin(q2R))/40564819207303340847894502572032 + (7514214926474921*sin(q2R)*((1917820484151683*cos(q1R))/18014398509481984 + (2579692110316253*sin(q1R))/4503599627370496))/36893488147419103232))/9007199254740992 - (106069577339469832923929692356850887620017617375*cos(q2R)*((1917820484151683*cos(q1R))/18014398509481984 + (2579692110316253*sin(q1R))/4503599627370496))/12554203470773361527671578846415332832204710888928069025792 + (14115856197532180673579726082375*sin(q2R)*((2579692110316253*cos(q1R))/4503599627370496 - (1917820484151683*sin(q1R))/18014398509481984))/340282366920938463463374607431768211456 + 323891950525769801103968238055131782751500431270071838086942675/231584178474632390847141970017375815706539969331281128078915168015826259279872))/9007199254740992 - (7514214926474921*cos(q5R)*((7514214926474921*cos(q4R)*((9007199067919185*cos(q3R)*((17274190877287359225804725738355*cos(q1R))/162259276829213363391578010288128 + (23235800371559029388956996013805*sin(q1R))/40564819207303340847894502572032 + 27504203825998033884751021716381/166153499473114484112975882535043072))/9007199254740992 - (7514214926474921*cos(q3R)*((32968958366167862000829996477285*cos(q2R))/40564819207303340847894502572032 - (7514214926474921*cos(q2R)*((1917820484151683*cos(q1R))/18014398509481984 + (2579692110316253*sin(q1R))/4503599627370496))/36893488147419103232 + sin(q2R)*((2579692110316253*cos(q1R))/4503599627370496 - (1917820484151683*sin(q1R))/18014398509481984)))/36893488147419103232 + sin(q3R)*(cos(q2R)*((2579692110316253*cos(q1R))/4503599627370496 - (1917820484151683*sin(q1R))/18014398509481984) - (32968958366167862000829996477285*sin(q2R))/40564819207303340847894502572032 + (7514214926474921*sin(q2R)*((1917820484151683*cos(q1R))/18014398509481984 + (2579692110316253*sin(q1R))/4503599627370496))/36893488147419103232)))/36893488147419103232 - ((4503599440548691*cos(q4R))/4503599627370496 - (7514214926474921*sin(q4R))/36893488147419103232)*(cos(q3R)*(cos(q2R)*((2579692110316253*cos(q1R))/4503599627370496 - (1917820484151683*sin(q1R))/18014398509481984) - (32968958366167862000829996477285*sin(q2R))/40564819207303340847894502572032 + (7514214926474921*sin(q2R)*((1917820484151683*cos(q1R))/18014398509481984 + (2579692110316253*sin(q1R))/4503599627370496))/36893488147419103232) - (9007199067919185*sin(q3R)*((17274190877287359225804725738355*cos(q1R))/162259276829213363391578010288128 + (23235800371559029388956996013805*sin(q1R))/40564819207303340847894502572032 + 27504203825998033884751021716381/166153499473114484112975882535043072))/9007199254740992 + (7514214926474921*sin(q3R)*((32968958366167862000829996477285*cos(q2R))/40564819207303340847894502572032 - (7514214926474921*cos(q2R)*((1917820484151683*cos(q1R))/18014398509481984 + (2579692110316253*sin(q1R))/4503599627370496))/36893488147419103232 + sin(q2R)*((2579692110316253*cos(q1R))/4503599627370496 - (1917820484151683*sin(q1R))/18014398509481984)))/36893488147419103232) + ((234819211581865*cos(q4R))/1152921504606846976 + (9007199067919185*sin(q4R))/9007199254740992)*((129801982932889585091297864435361917839115294955*cos(q1R))/5986310706507378352962293074805895248510699696029696 + (296957971066013582975066703729047659005068212725*cos(q2R))/365375409332725729550921208179070754913983135744 + (174598797980560374072834504815488878557302284405*sin(q1R))/1496577676626844588240573268701473812127674924007424 - (67682029681889335677290557259385*cos(q2R)*((1917820484151683*cos(q1R))/18014398509481984 + (2579692110316253*sin(q1R))/4503599627370496))/332306998946228968225951765070086144 + (9007199067919185*sin(q2R)*((2579692110316253*cos(q1R))/4503599627370496 - (1917820484151683*sin(q1R))/18014398509481984))/9007199254740992 + 206672498930123057048696703425560088887371380901/6129982163463555433433388108601236734474956488734408704)))/36893488147419103232 + sin(q5R)*(((7514214926474921*cos(q4R))/36893488147419103232 + (4503599440548691*sin(q4R))/4503599627370496)*(cos(q3R)*(cos(q2R)*((2579692110316253*cos(q1R))/4503599627370496 - (1917820484151683*sin(q1R))/18014398509481984) - (32968958366167862000829996477285*sin(q2R))/40564819207303340847894502572032 + (7514214926474921*sin(q2R)*((1917820484151683*cos(q1R))/18014398509481984 + (2579692110316253*sin(q1R))/4503599627370496))/36893488147419103232) - (9007199067919185*sin(q3R)*((17274190877287359225804725738355*cos(q1R))/162259276829213363391578010288128 + (23235800371559029388956996013805*sin(q1R))/40564819207303340847894502572032 + 27504203825998033884751021716381/166153499473114484112975882535043072))/9007199254740992 + (7514214926474921*sin(q3R)*((32968958366167862000829996477285*cos(q2R))/40564819207303340847894502572032 - (7514214926474921*cos(q2R)*((1917820484151683*cos(q1R))/18014398509481984 + (2579692110316253*sin(q1R))/4503599627370496))/36893488147419103232 + sin(q2R)*((2579692110316253*cos(q1R))/4503599627370496 - (1917820484151683*sin(q1R))/18014398509481984)))/36893488147419103232) - (7514214926474921*sin(q4R)*((9007199067919185*cos(q3R)*((17274190877287359225804725738355*cos(q1R))/162259276829213363391578010288128 + (23235800371559029388956996013805*sin(q1R))/40564819207303340847894502572032 + 27504203825998033884751021716381/166153499473114484112975882535043072))/9007199254740992 - (7514214926474921*cos(q3R)*((32968958366167862000829996477285*cos(q2R))/40564819207303340847894502572032 - (7514214926474921*cos(q2R)*((1917820484151683*cos(q1R))/18014398509481984 + (2579692110316253*sin(q1R))/4503599627370496))/36893488147419103232 + sin(q2R)*((2579692110316253*cos(q1R))/4503599627370496 - (1917820484151683*sin(q1R))/18014398509481984)))/36893488147419103232 + sin(q3R)*(cos(q2R)*((2579692110316253*cos(q1R))/4503599627370496 - (1917820484151683*sin(q1R))/18014398509481984) - (32968958366167862000829996477285*sin(q2R))/40564819207303340847894502572032 + (7514214926474921*sin(q2R)*((1917820484151683*cos(q1R))/18014398509481984 + (2579692110316253*sin(q1R))/4503599627370496))/36893488147419103232)))/36893488147419103232 + ((9007199067919185*cos(q4R))/9007199254740992 - (234819211581865*sin(q4R))/1152921504606846976)*((129801982932889585091297864435361917839115294955*cos(q1R))/5986310706507378352962293074805895248510699696029696 + (296957971066013582975066703729047659005068212725*cos(q2R))/365375409332725729550921208179070754913983135744 + (174598797980560374072834504815488878557302284405*sin(q1R))/1496577676626844588240573268701473812127674924007424 - (67682029681889335677290557259385*cos(q2R)*((1917820484151683*cos(q1R))/18014398509481984 + (2579692110316253*sin(q1R))/4503599627370496))/332306998946228968225951765070086144 + (9007199067919185*sin(q2R)*((2579692110316253*cos(q1R))/4503599627370496 - (1917820484151683*sin(q1R))/18014398509481984))/9007199254740992 + 206672498930123057048696703425560088887371380901/6129982163463555433433388108601236734474956488734408704))))/1000 + (2436553109258773196144549622003023*cos(q6R)*(cos(q5R)*(((7514214926474921*cos(q4R))/36893488147419103232 + (4503599440548691*sin(q4R))/4503599627370496)*(cos(q3R)*(cos(q2R)*((2579692110316253*cos(q1R))/4503599627370496 - (1917820484151683*sin(q1R))/18014398509481984) - (32968958366167862000829996477285*sin(q2R))/40564819207303340847894502572032 + (7514214926474921*sin(q2R)*((1917820484151683*cos(q1R))/18014398509481984 + (2579692110316253*sin(q1R))/4503599627370496))/36893488147419103232) - (9007199067919185*sin(q3R)*((17274190877287359225804725738355*cos(q1R))/162259276829213363391578010288128 + (23235800371559029388956996013805*sin(q1R))/40564819207303340847894502572032 + 27504203825998033884751021716381/166153499473114484112975882535043072))/9007199254740992 + (7514214926474921*sin(q3R)*((32968958366167862000829996477285*cos(q2R))/40564819207303340847894502572032 - (7514214926474921*cos(q2R)*((1917820484151683*cos(q1R))/18014398509481984 + (2579692110316253*sin(q1R))/4503599627370496))/36893488147419103232 + sin(q2R)*((2579692110316253*cos(q1R))/4503599627370496 - (1917820484151683*sin(q1R))/18014398509481984)))/36893488147419103232) - (7514214926474921*sin(q4R)*((9007199067919185*cos(q3R)*((17274190877287359225804725738355*cos(q1R))/162259276829213363391578010288128 + (23235800371559029388956996013805*sin(q1R))/40564819207303340847894502572032 + 27504203825998033884751021716381/166153499473114484112975882535043072))/9007199254740992 - (7514214926474921*cos(q3R)*((32968958366167862000829996477285*cos(q2R))/40564819207303340847894502572032 - (7514214926474921*cos(q2R)*((1917820484151683*cos(q1R))/18014398509481984 + (2579692110316253*sin(q1R))/4503599627370496))/36893488147419103232 + sin(q2R)*((2579692110316253*cos(q1R))/4503599627370496 - (1917820484151683*sin(q1R))/18014398509481984)))/36893488147419103232 + sin(q3R)*(cos(q2R)*((2579692110316253*cos(q1R))/4503599627370496 - (1917820484151683*sin(q1R))/18014398509481984) - (32968958366167862000829996477285*sin(q2R))/40564819207303340847894502572032 + (7514214926474921*sin(q2R)*((1917820484151683*cos(q1R))/18014398509481984 + (2579692110316253*sin(q1R))/4503599627370496))/36893488147419103232)))/36893488147419103232 + ((9007199067919185*cos(q4R))/9007199254740992 - (234819211581865*sin(q4R))/1152921504606846976)*((129801982932889585091297864435361917839115294955*cos(q1R))/5986310706507378352962293074805895248510699696029696 + (296957971066013582975066703729047659005068212725*cos(q2R))/365375409332725729550921208179070754913983135744 + (174598797980560374072834504815488878557302284405*sin(q1R))/1496577676626844588240573268701473812127674924007424 - (67682029681889335677290557259385*cos(q2R)*((1917820484151683*cos(q1R))/18014398509481984 + (2579692110316253*sin(q1R))/4503599627370496))/332306998946228968225951765070086144 + (9007199067919185*sin(q2R)*((2579692110316253*cos(q1R))/4503599627370496 - (1917820484151683*sin(q1R))/18014398509481984))/9007199254740992 + 206672498930123057048696703425560088887371380901/6129982163463555433433388108601236734474956488734408704)) - (9007199067919185*sin(q5R)*((203422408166946418981152780445187297537016008229516441756292125*cos(q1R))/226156424291633194186662080095093570025917938800079226639565593765455331328 + (465385075279251052437186083221547446448384963368966483726351875*cos(q2R))/13803492693581127574869511724554050904902217944340773110325048447598592 + (273626851807209941619219010639387076236787289365779842797695875*sin(q1R))/56539106072908298546665520023773392506479484700019806659891398441363832832 - (81129635049124235038645691064225*cos(q3R)*((17274190877287359225804725738355*cos(q1R))/162259276829213363391578010288128 + (23235800371559029388956996013805*sin(q1R))/40564819207303340847894502572032 + 27504203825998033884751021716381/166153499473114484112975882535043072))/81129638414606681695789005144064 + (2115063383689692319117831580025*sin(q3R)*((17274190877287359225804725738355*cos(q1R))/162259276829213363391578010288128 + (23235800371559029388956996013805*sin(q1R))/40564819207303340847894502572032 + 27504203825998033884751021716381/166153499473114484112975882535043072))/10384593717069655257060992658440192 + (67682029681889335677290557259385*cos(q3R)*((32968958366167862000829996477285*cos(q2R))/40564819207303340847894502572032 - (7514214926474921*cos(q2R)*((1917820484151683*cos(q1R))/18014398509481984 + (2579692110316253*sin(q1R))/4503599627370496))/36893488147419103232 + sin(q2R)*((2579692110316253*cos(q1R))/4503599627370496 - (1917820484151683*sin(q1R))/18014398509481984)))/332306998946228968225951765070086144 - (234819211581865*cos(q3R)*(cos(q2R)*((2579692110316253*cos(q1R))/4503599627370496 - (1917820484151683*sin(q1R))/18014398509481984) - (32968958366167862000829996477285*sin(q2R))/40564819207303340847894502572032 + (7514214926474921*sin(q2R)*((1917820484151683*cos(q1R))/18014398509481984 + (2579692110316253*sin(q1R))/4503599627370496))/36893488147419103232))/1152921504606846976 - (1764482024691522628700660907665*sin(q3R)*((32968958366167862000829996477285*cos(q2R))/40564819207303340847894502572032 - (7514214926474921*cos(q2R)*((1917820484151683*cos(q1R))/18014398509481984 + (2579692110316253*sin(q1R))/4503599627370496))/36893488147419103232 + sin(q2R)*((2579692110316253*cos(q1R))/4503599627370496 - (1917820484151683*sin(q1R))/18014398509481984)))/42535295865117307932921825928971026432 - (9007199067919185*sin(q3R)*(cos(q2R)*((2579692110316253*cos(q1R))/4503599627370496 - (1917820484151683*sin(q1R))/18014398509481984) - (32968958366167862000829996477285*sin(q2R))/40564819207303340847894502572032 + (7514214926474921*sin(q2R)*((1917820484151683*cos(q1R))/18014398509481984 + (2579692110316253*sin(q1R))/4503599627370496))/36893488147419103232))/9007199254740992 - (106069577339469832923929692356850887620017617375*cos(q2R)*((1917820484151683*cos(q1R))/18014398509481984 + (2579692110316253*sin(q1R))/4503599627370496))/12554203470773361527671578846415332832204710888928069025792 + (14115856197532180673579726082375*sin(q2R)*((2579692110316253*cos(q1R))/4503599627370496 - (1917820484151683*sin(q1R))/18014398509481984))/340282366920938463463374607431768211456 + 323891950525769801103968238055131782751500431270071838086942675/231584178474632390847141970017375815706539969331281128078915168015826259279872))/9007199254740992 + (7514214926474921*sin(q5R)*((7514214926474921*cos(q4R)*((9007199067919185*cos(q3R)*((17274190877287359225804725738355*cos(q1R))/162259276829213363391578010288128 + (23235800371559029388956996013805*sin(q1R))/40564819207303340847894502572032 + 27504203825998033884751021716381/166153499473114484112975882535043072))/9007199254740992 - (7514214926474921*cos(q3R)*((32968958366167862000829996477285*cos(q2R))/40564819207303340847894502572032 - (7514214926474921*cos(q2R)*((1917820484151683*cos(q1R))/18014398509481984 + (2579692110316253*sin(q1R))/4503599627370496))/36893488147419103232 + sin(q2R)*((2579692110316253*cos(q1R))/4503599627370496 - (1917820484151683*sin(q1R))/18014398509481984)))/36893488147419103232 + sin(q3R)*(cos(q2R)*((2579692110316253*cos(q1R))/4503599627370496 - (1917820484151683*sin(q1R))/18014398509481984) - (32968958366167862000829996477285*sin(q2R))/40564819207303340847894502572032 + (7514214926474921*sin(q2R)*((1917820484151683*cos(q1R))/18014398509481984 + (2579692110316253*sin(q1R))/4503599627370496))/36893488147419103232)))/36893488147419103232 - ((4503599440548691*cos(q4R))/4503599627370496 - (7514214926474921*sin(q4R))/36893488147419103232)*(cos(q3R)*(cos(q2R)*((2579692110316253*cos(q1R))/4503599627370496 - (1917820484151683*sin(q1R))/18014398509481984) - (32968958366167862000829996477285*sin(q2R))/40564819207303340847894502572032 + (7514214926474921*sin(q2R)*((1917820484151683*cos(q1R))/18014398509481984 + (2579692110316253*sin(q1R))/4503599627370496))/36893488147419103232) - (9007199067919185*sin(q3R)*((17274190877287359225804725738355*cos(q1R))/162259276829213363391578010288128 + (23235800371559029388956996013805*sin(q1R))/40564819207303340847894502572032 + 27504203825998033884751021716381/166153499473114484112975882535043072))/9007199254740992 + (7514214926474921*sin(q3R)*((32968958366167862000829996477285*cos(q2R))/40564819207303340847894502572032 - (7514214926474921*cos(q2R)*((1917820484151683*cos(q1R))/18014398509481984 + (2579692110316253*sin(q1R))/4503599627370496))/36893488147419103232 + sin(q2R)*((2579692110316253*cos(q1R))/4503599627370496 - (1917820484151683*sin(q1R))/18014398509481984)))/36893488147419103232) + ((234819211581865*cos(q4R))/1152921504606846976 + (9007199067919185*sin(q4R))/9007199254740992)*((129801982932889585091297864435361917839115294955*cos(q1R))/5986310706507378352962293074805895248510699696029696 + (296957971066013582975066703729047659005068212725*cos(q2R))/365375409332725729550921208179070754913983135744 + (174598797980560374072834504815488878557302284405*sin(q1R))/1496577676626844588240573268701473812127674924007424 - (67682029681889335677290557259385*cos(q2R)*((1917820484151683*cos(q1R))/18014398509481984 + (2579692110316253*sin(q1R))/4503599627370496))/332306998946228968225951765070086144 + (9007199067919185*sin(q2R)*((2579692110316253*cos(q1R))/4503599627370496 - (1917820484151683*sin(q1R))/18014398509481984))/9007199254740992 + 206672498930123057048696703425560088887371380901/6129982163463555433433388108601236734474956488734408704)))/36893488147419103232))/332306998946228968225951765070086144000 + (324259171862923063*sin(q6R)*((9007199067919185*cos(q5R)*((203422408166946418981152780445187297537016008229516441756292125*cos(q1R))/226156424291633194186662080095093570025917938800079226639565593765455331328 + (465385075279251052437186083221547446448384963368966483726351875*cos(q2R))/13803492693581127574869511724554050904902217944340773110325048447598592 + (273626851807209941619219010639387076236787289365779842797695875*sin(q1R))/56539106072908298546665520023773392506479484700019806659891398441363832832 - (81129635049124235038645691064225*cos(q3R)*((17274190877287359225804725738355*cos(q1R))/162259276829213363391578010288128 + (23235800371559029388956996013805*sin(q1R))/40564819207303340847894502572032 + 27504203825998033884751021716381/166153499473114484112975882535043072))/81129638414606681695789005144064 + (2115063383689692319117831580025*sin(q3R)*((17274190877287359225804725738355*cos(q1R))/162259276829213363391578010288128 + (23235800371559029388956996013805*sin(q1R))/40564819207303340847894502572032 + 27504203825998033884751021716381/166153499473114484112975882535043072))/10384593717069655257060992658440192 + (67682029681889335677290557259385*cos(q3R)*((32968958366167862000829996477285*cos(q2R))/40564819207303340847894502572032 - (7514214926474921*cos(q2R)*((1917820484151683*cos(q1R))/18014398509481984 + (2579692110316253*sin(q1R))/4503599627370496))/36893488147419103232 + sin(q2R)*((2579692110316253*cos(q1R))/4503599627370496 - (1917820484151683*sin(q1R))/18014398509481984)))/332306998946228968225951765070086144 - (234819211581865*cos(q3R)*(cos(q2R)*((2579692110316253*cos(q1R))/4503599627370496 - (1917820484151683*sin(q1R))/18014398509481984) - (32968958366167862000829996477285*sin(q2R))/40564819207303340847894502572032 + (7514214926474921*sin(q2R)*((1917820484151683*cos(q1R))/18014398509481984 + (2579692110316253*sin(q1R))/4503599627370496))/36893488147419103232))/1152921504606846976 - (1764482024691522628700660907665*sin(q3R)*((32968958366167862000829996477285*cos(q2R))/40564819207303340847894502572032 - (7514214926474921*cos(q2R)*((1917820484151683*cos(q1R))/18014398509481984 + (2579692110316253*sin(q1R))/4503599627370496))/36893488147419103232 + sin(q2R)*((2579692110316253*cos(q1R))/4503599627370496 - (1917820484151683*sin(q1R))/18014398509481984)))/42535295865117307932921825928971026432 - (9007199067919185*sin(q3R)*(cos(q2R)*((2579692110316253*cos(q1R))/4503599627370496 - (1917820484151683*sin(q1R))/18014398509481984) - (32968958366167862000829996477285*sin(q2R))/40564819207303340847894502572032 + (7514214926474921*sin(q2R)*((1917820484151683*cos(q1R))/18014398509481984 + (2579692110316253*sin(q1R))/4503599627370496))/36893488147419103232))/9007199254740992 - (106069577339469832923929692356850887620017617375*cos(q2R)*((1917820484151683*cos(q1R))/18014398509481984 + (2579692110316253*sin(q1R))/4503599627370496))/12554203470773361527671578846415332832204710888928069025792 + (14115856197532180673579726082375*sin(q2R)*((2579692110316253*cos(q1R))/4503599627370496 - (1917820484151683*sin(q1R))/18014398509481984))/340282366920938463463374607431768211456 + 323891950525769801103968238055131782751500431270071838086942675/231584178474632390847141970017375815706539969331281128078915168015826259279872))/9007199254740992 - (7514214926474921*cos(q5R)*((7514214926474921*cos(q4R)*((9007199067919185*cos(q3R)*((17274190877287359225804725738355*cos(q1R))/162259276829213363391578010288128 + (23235800371559029388956996013805*sin(q1R))/40564819207303340847894502572032 + 27504203825998033884751021716381/166153499473114484112975882535043072))/9007199254740992 - (7514214926474921*cos(q3R)*((32968958366167862000829996477285*cos(q2R))/40564819207303340847894502572032 - (7514214926474921*cos(q2R)*((1917820484151683*cos(q1R))/18014398509481984 + (2579692110316253*sin(q1R))/4503599627370496))/36893488147419103232 + sin(q2R)*((2579692110316253*cos(q1R))/4503599627370496 - (1917820484151683*sin(q1R))/18014398509481984)))/36893488147419103232 + sin(q3R)*(cos(q2R)*((2579692110316253*cos(q1R))/4503599627370496 - (1917820484151683*sin(q1R))/18014398509481984) - (32968958366167862000829996477285*sin(q2R))/40564819207303340847894502572032 + (7514214926474921*sin(q2R)*((1917820484151683*cos(q1R))/18014398509481984 + (2579692110316253*sin(q1R))/4503599627370496))/36893488147419103232)))/36893488147419103232 - ((4503599440548691*cos(q4R))/4503599627370496 - (7514214926474921*sin(q4R))/36893488147419103232)*(cos(q3R)*(cos(q2R)*((2579692110316253*cos(q1R))/4503599627370496 - (1917820484151683*sin(q1R))/18014398509481984) - (32968958366167862000829996477285*sin(q2R))/40564819207303340847894502572032 + (7514214926474921*sin(q2R)*((1917820484151683*cos(q1R))/18014398509481984 + (2579692110316253*sin(q1R))/4503599627370496))/36893488147419103232) - (9007199067919185*sin(q3R)*((17274190877287359225804725738355*cos(q1R))/162259276829213363391578010288128 + (23235800371559029388956996013805*sin(q1R))/40564819207303340847894502572032 + 27504203825998033884751021716381/166153499473114484112975882535043072))/9007199254740992 + (7514214926474921*sin(q3R)*((32968958366167862000829996477285*cos(q2R))/40564819207303340847894502572032 - (7514214926474921*cos(q2R)*((1917820484151683*cos(q1R))/18014398509481984 + 